simulink model "Speedmeter_harness"  (R2019b)
settings: Solver=FixedStepDiscrete  StartTime=0  StopTime=0.58999999999999997  FixedStep=0.01  RelTol=1e-3
undefined symbols (not defined in the file): Const16_0, Const16_2, Const16_210, Const16_340, Const16_350, Const16_4, Const8_0, Const8_1, Const8_2, Const8_4, ConstFL_00879, ConstFL_01, ConstFL_03516, ConstFL_1_6093, sigbuilder_block, STEP_TIME
libraries: simulink x2
(part 1 of 2)
settings Model: DataTypeOverride=Single  SldvGeneratedHarnessModel=TestUnitModel=Speedmeter|  ModifiedByFormat=TATA ELXSI LTD  Creator=TATA ELXSI LTD  LastModifiedBy=TATA ELXSI LTD
settings ConfigSet: Description=Test1
settings DataIOCC: LimitDataPoints=on  SaveFormat=StructureWithTime  ReturnWorkspaceOutputs=off
settings OptimizationCC: BlockReduction=off  ExpressionFolding=off  LifeSpan=inf
settings DebuggingCC: UnderspecifiedInitializationDetection=Classic  MergeDetectMultiDrivingBlocksExec=none  SolverPrmCheckMsg=warning  InheritedTsInSrcMsg=none  ParameterPrecisionLossMsg=none  FcnCallInpInsideContextMsg=warning  StateNameClashWarn=warning  SFUnexpectedBacktrackingDiag=warning  SFNoUnconditionalDefaultTransitionDiag=warning  SFExecutionAtInitializationDiag=none
settings HardwareCC: ProdBitPerPointer=32  ProdBitPerSizeT=32  ProdBitPerPtrDiffT=32  ProdLargestAtomicFloat=None  ProdWordSize=32  ProdHWDeviceType=Generic->32-bit x86 compatible
settings ModelReferenceCC: PropagateSignalLabelsOutOfModel=off
settings RTWCC: Description=Generic Real-Time Target
settings CodeAppCC: StateflowObjectComments=on
settings GRTTargetCC: TargetLangStandard=C89/C90 (ANSI)  CombineOutputUpdateFcns=off  GRTInterface=on
settings ConfigComp: CovEnable=on  RecordCoverage=on  CovMetricSettings=dcmo  CovHTMLOptions=-aTS=1 -bRG=1 -bTC=0 -hTR=0 -nFC=0 -scm=1 -bcm=1  CovHtmlReporting=on  CovSaveCumulativeToWorkspaceVar=on  CovCumulativeReport=on  CovShowResultsExplorer=off  CovModelRefEnable=on  DVMaxTestCaseSteps=500  DVTestSuiteOptimization=CombinedObjectives (Nonlinear Extended)  DVDetectDeadLogic=on  DVDetectActiveLogic=on  DVDetectOutOfBounds=on

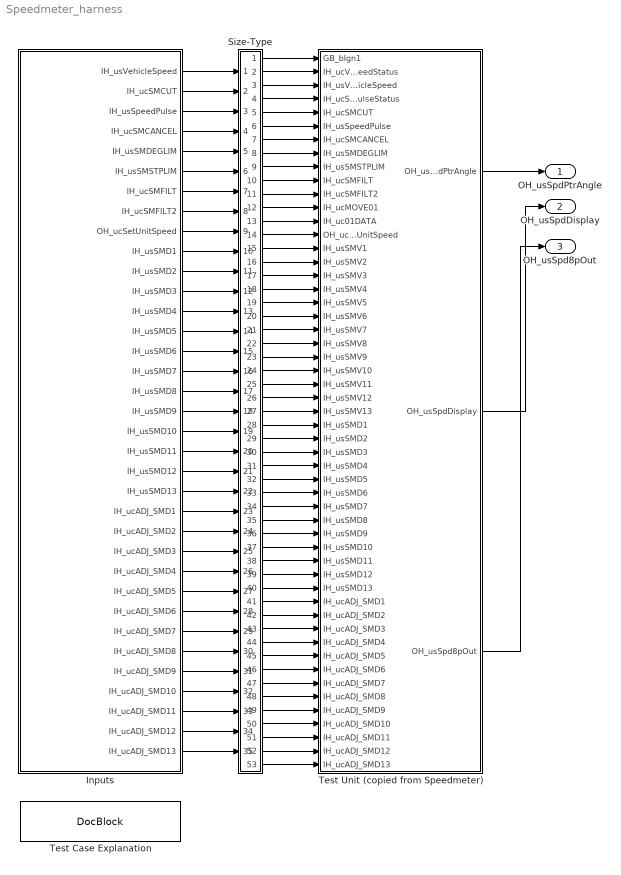
== system Speedmeter_harness ==
  Inputs : Subsystem  Tag=STV Subsys  LoadFcn=sigbuilder_block('load',[50 50 520 400 ]);  StartFcn=sigbuilder_block('start');  StopFcn=sigbuilder_block('stop');  ClipboardFcn=sigbuilder_block('clipboard');  mask(Sigbuilder block){tuvar=[0:10]}
      mask init:
      | if ~strcmp(get_param(bdroot(gcb),'SimulationStatus'),'stopped'),tuvar = sigbuilder_block('maskInit'); end
      settings: CopyFcn=sigbuilder_block('copy');  DeleteFcn=sigbuilder_block('delete');  ModelCloseFcn=sigbuilder_block('modelClose');  PreSaveFcn=sigbuilder_block('preSave');  PauseFcn=sigbuilder_block('pause');  ContinueFcn=sigbuilder_block('continue');  NameChangeFcn=sigbuilder_block('namechange');  OpenFcn=sigbuilder_block('open');  CloseFcn=sigbuilder_block('close');
      mask Display: plot(0, 0, 100, 100,[2, 2, 32, 32, 2], [68, 8, 8, 68, 68],[32, 2], [38, 38], [32, 19, 2],[53, 60, 44], [32, 17, 17, 2],[16, 16, 31, 31]);txt = getActiveGroup(gcbh);text(2, 100, txt,'verticalAlignment', 'top');
  Size-Type : Subsystem
  Test Case Explanation : simulink/Model-Wide Utilities/DocBlock  DocumentType=Text
  Test Unit (copied from Speedmeter) : Subsystem
  OH_usSpdPtrAngle : Outport  OutMin=0  OutMax=4095  OutDataTypeStr=fixdt(0,16,0.0879,0)  SampleTime=STEP_TIME  VectorParamsAs1DForOutWhenUnconnected=off
  OH_usSpdDisplay : Outport  Port=2  OutDataTypeStr=fixdt(0,16,1,0)  SampleTime=STEP_TIME  VectorParamsAs1DForOutWhenUnconnected=off
  OH_usSpd8pOut : Outport  Port=3  OutMin=0  OutMax=655.34  OutDataTypeStr=fixdt(0,16,0.01,0)  SampleTime=STEP_TIME  VectorParamsAs1DForOutWhenUnconnected=off
  wires:
  Size-Type/1(Out1) -> Test Unit (copied from Speedmeter)/1(GB_bIgn1)
  Size-Type/2(Out2) -> Test Unit (copied from Speedmeter)/2(IH_ucVehicleSpeedStatus)
  Inputs/1(IH_usVehicleSpeed) -> Size-Type/1(In3)
  Size-Type/3(Out3) -> Test Unit (copied from Speedmeter)/3(IH_usVehicleSpeed)
  Size-Type/4(Out4) -> Test Unit (copied from Speedmeter)/4(IH_ucSpeedPulseStatus)
  Inputs/2(IH_ucSMCUT) -> Size-Type/2(In5)
  Size-Type/5(Out5) -> Test Unit (copied from Speedmeter)/5(IH_ucSMCUT)
  Inputs/3(IH_usSpeedPulse) -> Size-Type/3(In6)
  Size-Type/6(Out6) -> Test Unit (copied from Speedmeter)/6(IH_usSpeedPulse)
  Inputs/4(IH_ucSMCANCEL) -> Size-Type/4(In7)
  Size-Type/7(Out7) -> Test Unit (copied from Speedmeter)/7(IH_ucSMCANCEL)
  Inputs/5(IH_usSMDEGLIM) -> Size-Type/5(In8)
  Size-Type/8(Out8) -> Test Unit (copied from Speedmeter)/8(IH_usSMDEGLIM)
  Inputs/6(IH_usSMSTPLIM) -> Size-Type/6(In9)
  Size-Type/9(Out9) -> Test Unit (copied from Speedmeter)/9(IH_usSMSTPLIM)
  Inputs/7(IH_ucSMFILT) -> Size-Type/7(In10)
  Size-Type/10(Out10) -> Test Unit (copied from Speedmeter)/10(IH_ucSMFILT)
  Inputs/8(IH_ucSMFILT2) -> Size-Type/8(In11)
  Size-Type/11(Out11) -> Test Unit (copied from Speedmeter)/11(IH_ucSMFILT2)
  Size-Type/12(Out12) -> Test Unit (copied from Speedmeter)/12(IH_ucMOVE01)
  Size-Type/13(Out13) -> Test Unit (copied from Speedmeter)/13(IH_uc01DATA)
  Inputs/9(OH_ucSetUnitSpeed) -> Size-Type/9(In14)
  Size-Type/14(Out14) -> Test Unit (copied from Speedmeter)/14(OH_ucSetUnitSpeed)
  Size-Type/15(Out15) -> Test Unit (copied from Speedmeter)/15(IH_usSMV1)
  Size-Type/16(Out16) -> Test Unit (copied from Speedmeter)/16(IH_usSMV2)
  Size-Type/17(Out17) -> Test Unit (copied from Speedmeter)/17(IH_usSMV3)
  Size-Type/18(Out18) -> Test Unit (copied from Speedmeter)/18(IH_usSMV4)
  Size-Type/19(Out19) -> Test Unit (copied from Speedmeter)/19(IH_usSMV5)
  Size-Type/20(Out20) -> Test Unit (copied from Speedmeter)/20(IH_usSMV6)
  Size-Type/21(Out21) -> Test Unit (copied from Speedmeter)/21(IH_usSMV7)
  Size-Type/22(Out22) -> Test Unit (copied from Speedmeter)/22(IH_usSMV8)
  Size-Type/23(Out23) -> Test Unit (copied from Speedmeter)/23(IH_usSMV9)
  Size-Type/24(Out24) -> Test Unit (copied from Speedmeter)/24(IH_usSMV10)
  Size-Type/25(Out25) -> Test Unit (copied from Speedmeter)/25(IH_usSMV11)
  Size-Type/26(Out26) -> Test Unit (copied from Speedmeter)/26(IH_usSMV12)
  Size-Type/27(Out27) -> Test Unit (copied from Speedmeter)/27(IH_usSMV13)
  Inputs/10(IH_usSMD1) -> Size-Type/10(In28)
  Size-Type/28(Out28) -> Test Unit (copied from Speedmeter)/28(IH_usSMD1)
  Inputs/11(IH_usSMD2) -> Size-Type/11(In29)
  Size-Type/29(Out29) -> Test Unit (copied from Speedmeter)/29(IH_usSMD2)
  Inputs/12(IH_usSMD3) -> Size-Type/12(In30)
  Size-Type/30(Out30) -> Test Unit (copied from Speedmeter)/30(IH_usSMD3)
  Inputs/13(IH_usSMD4) -> Size-Type/13(In31)
  Size-Type/31(Out31) -> Test Unit (copied from Speedmeter)/31(IH_usSMD4)
  Inputs/14(IH_usSMD5) -> Size-Type/14(In32)
  Size-Type/32(Out32) -> Test Unit (copied from Speedmeter)/32(IH_usSMD5)
  Inputs/15(IH_usSMD6) -> Size-Type/15(In33)
  Size-Type/33(Out33) -> Test Unit (copied from Speedmeter)/33(IH_usSMD6)
  Inputs/16(IH_usSMD7) -> Size-Type/16(In34)
  Size-Type/34(Out34) -> Test Unit (copied from Speedmeter)/34(IH_usSMD7)
  Inputs/17(IH_usSMD8) -> Size-Type/17(In35)
  Size-Type/35(Out35) -> Test Unit (copied from Speedmeter)/35(IH_usSMD8)
  Inputs/18(IH_usSMD9) -> Size-Type/18(In36)
  Size-Type/36(Out36) -> Test Unit (copied from Speedmeter)/36(IH_usSMD9)
  Inputs/19(IH_usSMD10) -> Size-Type/19(In37)
  Size-Type/37(Out37) -> Test Unit (copied from Speedmeter)/37(IH_usSMD10)
  Inputs/20(IH_usSMD11) -> Size-Type/20(In38)
  Size-Type/38(Out38) -> Test Unit (copied from Speedmeter)/38(IH_usSMD11)
  Inputs/21(IH_usSMD12) -> Size-Type/21(In39)
  Size-Type/39(Out39) -> Test Unit (copied from Speedmeter)/39(IH_usSMD12)
  Inputs/22(IH_usSMD13) -> Size-Type/22(In40)
  Size-Type/40(Out40) -> Test Unit (copied from Speedmeter)/40(IH_usSMD13)
  Inputs/23(IH_ucADJ_SMD1) -> Size-Type/23(In41)
  Size-Type/41(Out41) -> Test Unit (copied from Speedmeter)/41(IH_ucADJ_SMD1)
  Inputs/24(IH_ucADJ_SMD2) -> Size-Type/24(In42)
  Size-Type/42(Out42) -> Test Unit (copied from Speedmeter)/42(IH_ucADJ_SMD2)
  Inputs/25(IH_ucADJ_SMD3) -> Size-Type/25(In43)
  Size-Type/43(Out43) -> Test Unit (copied from Speedmeter)/43(IH_ucADJ_SMD3)
  Inputs/26(IH_ucADJ_SMD4) -> Size-Type/26(In44)
  Size-Type/44(Out44) -> Test Unit (copied from Speedmeter)/44(IH_ucADJ_SMD4)
  Inputs/27(IH_ucADJ_SMD5) -> Size-Type/27(In45)
  Size-Type/45(Out45) -> Test Unit (copied from Speedmeter)/45(IH_ucADJ_SMD5)
  Inputs/28(IH_ucADJ_SMD6) -> Size-Type/28(In46)
  Size-Type/46(Out46) -> Test Unit (copied from Speedmeter)/46(IH_ucADJ_SMD6)
  Inputs/29(IH_ucADJ_SMD7) -> Size-Type/29(In47)
  Size-Type/47(Out47) -> Test Unit (copied from Speedmeter)/47(IH_ucADJ_SMD7)
  Inputs/30(IH_ucADJ_SMD8) -> Size-Type/30(In48)
  Size-Type/48(Out48) -> Test Unit (copied from Speedmeter)/48(IH_ucADJ_SMD8)
  Inputs/31(IH_ucADJ_SMD9) -> Size-Type/31(In49)
  Size-Type/49(Out49) -> Test Unit (copied from Speedmeter)/49(IH_ucADJ_SMD9)
  Inputs/32(IH_ucADJ_SMD10) -> Size-Type/32(In50)
  Size-Type/50(Out50) -> Test Unit (copied from Speedmeter)/50(IH_ucADJ_SMD10)
  Inputs/33(IH_ucADJ_SMD11) -> Size-Type/33(In51)
  Size-Type/51(Out51) -> Test Unit (copied from Speedmeter)/51(IH_ucADJ_SMD11)
  Inputs/34(IH_ucADJ_SMD12) -> Size-Type/34(In52)
  Size-Type/52(Out52) -> Test Unit (copied from Speedmeter)/52(IH_ucADJ_SMD12)
  Inputs/35(IH_ucADJ_SMD13) -> Size-Type/35(In53)
  Size-Type/53(Out53) -> Test Unit (copied from Speedmeter)/53(IH_ucADJ_SMD13)
  Test Unit (copied from Speedmeter)/1(OH_usSpdPtrAngle) -> OH_usSpdPtrAngle/1
  Test Unit (copied from Speedmeter)/2(OH_usSpdDisplay) -> OH_usSpdDisplay/1
  Test Unit (copied from Speedmeter)/3(OH_usSpd8pOut) -> OH_usSpd8pOut/1

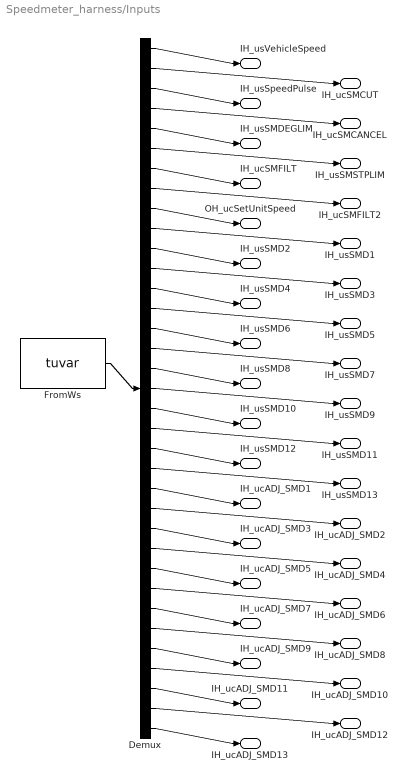
== system Speedmeter_harness/Inputs ==
  Demux : Demux  Tag=STV Demux  Outputs=35
  FromWs : FromWorkspace  Tag=STV FromWs  VariableName=tuvar  SampleTime=0
      SigBuilderData=|
      | dataSet.timeRange = [0 2.38]
      | dataSet.name = 'Test Case 1'
      | sbobj.Name = 'Signal Builder'
      | sbobj.Groups.Name = 'Test Case 1'
      | sbobj.Groups.Signals(1).Name = 'IH_usVehicleSpeed'
      | sbobj.Groups.Signals(1).XData = [0 2.18 2.18 2.21 2.23 2.35 2.36 2.37 2.38]
      | sbobj.Groups.Signals(1).YData = [404.191131592 404.191131592 0 0 0 0 0 0 0]
      | sbobj.Groups.Signals(2).Name = 'IH_ucSMCUT'
      | sbobj.Groups.Signals(2).XData = [0 2.18 2.18 2.21 2.23 2.35 2.36 2.37 2.38]
      | sbobj.Groups.Signals(2).YData = [1.79223001003 1.79223001003 0 0 0 0 0 0 0]
      | sbobj.Groups.Signals(3).Name = 'IH_usSpeedPulse'
      | sbobj.Groups.Signals(3).XData = [0 2.18 2.18 2.21 2.21 2.23 2.23 2.35 2.35 2.36 2.36 2.37 2.38]
      | sbobj.Groups.Signals(3).YData = [320.146972656 320.146972656 0 0 655.349975586 655.349975586 0 0 655.349975586 655.349975586 0 0 0]
      | sbobj.Groups.Signals(4).Name = 'IH_ucSMCANCEL'
      | sbobj.Groups.Signals(4).XData = [0 2.18 2.18 2.21 2.23 2.35 2.36 2.37 2.37 2.38]
      | sbobj.Groups.Signals(4).YData = [1.19769001007 1.19769001007 0 0 0 0 0 0 10.899600029 10.899600029]
      | sbobj.Groups.Signals(5).Name = 'IH_usSMDEGLIM'
      | sbobj.Groups.Signals(5).XData = [0 2.18 2.21 2.23 2.35 2.35 2.36 2.36 2.37 2.38]
      | sbobj.Groups.Signals(5).YData = [140.597106934 140.597106934 140.597106934 140.597106934 140.597106934 82.1601867676 82.1601867676 0 0 0]
      | sbobj.Groups.Signals(6).Name = 'IH_usSMSTPLIM'
      | sbobj.Groups.Signals(6).XData = [0 2.18 2.18 2.21 2.23 2.35 2.35 2.36 2.37 2.38]
      | sbobj.Groups.Signals(6).YData = [0.951390028 0.951390028 5.53770017624 5.53770017624 5.53770017624 5.53770017624 0 0 0 0]
      | sbobj.Groups.Signals(7).Name = 'IH_ucSMFILT'
      | sbobj.Groups.Signals(7).XData = [0 2.18 2.21 2.23 2.35 2.36 2.37 2.37 2.38]
      | sbobj.Groups.Signals(7).YData = [4.00516986847 4.00516986847 4.00516986847 4.00516986847 4.00516986847 4.00516986847 4.00516986847 0 0]
      | sbobj.Groups.Signals(8).Name = 'IH_ucSMFILT2'
      | sbobj.Groups.Signals(8).XData = [0 2.18 2.21 2.23 2.35 2.36 2.37 2.37 2.38]
      | sbobj.Groups.Signals(8).YData = [1.31280994415 1.31280994415 1.31280994415 1.31280994415 1.31280994415 1.31280994415 1.31280994415 0 0]
      | sbobj.Groups.Signals(9).Name = 'OH_ucSetUnitSpeed'
      | sbobj.Groups.Signals(9).XData = [0 2.18 2.18 2.21 2.23 2.23 2.35 2.36 2.36 2.37 2.38]
      | sbobj.Groups.Signals(9).YData = [0.490040004253 0.490040004253 0 0 0 1 1 1 0 0 0]
      | sbobj.Groups.Signals(10).Name = 'IH_usSMD1'
      | sbobj.Groups.Signals(10).XData = [0 2.18 2.18 2.21 2.23 2.35 2.36 2.37 2.38]
      | sbobj.Groups.Signals(10).YData = [192.551025391 192.551025391 0 0 0 0 0 0 0]
      | sbobj.Groups.Signals(11).Name = 'IH_usSMD2'
      | sbobj.Groups.Signals(11).XData = [0 2.18 2.18 2.21 2.23 2.35 2.35 2.36 2.36 2.37 2.38]
      | sbobj.Groups.Signals(11).YData = [115.773422241 115.773422241 0 0 0 0 359.950500488 359.950500488 0 0 0]
      | sbobj.Groups.Signals(12).Name = 'IH_usSMD3'
      | sbobj.Groups.Signals(12).XData = [0 2.18 2.18 2.21 2.23 2.35 2.35 2.36 2.36 2.37 2.38]
      | sbobj.Groups.Signals(12).YData = [191.705841064 191.705841064 0 0 0 0 359.950500488 359.950500488 0 0 0]
      | sbobj.Groups.Signals(13).Name = 'IH_usSMD4'
      | sbobj.Groups.Signals(13).XData = [0 2.18 2.18 2.21 2.23 2.35 2.35 2.36 2.36 2.37 2.38]
      | sbobj.Groups.Signals(13).YData = [73.4985580444 73.4985580444 0 0 0 0 359.950500488 359.950500488 0 0 0]
      | sbobj.Groups.Signals(14).Name = 'IH_usSMD5'
      | sbobj.Groups.Signals(14).XData = [0 2.18 2.18 2.21 2.23 2.35 2.35 2.36 2.36 2.37 2.38]
      | sbobj.Groups.Signals(14).YData = [124.571632385 124.571632385 0 0 0 0 359.950500488 359.950500488 0 0 0]
      | sbobj.Groups.Signals(15).Name = 'IH_usSMD6'
      | sbobj.Groups.Signals(15).XData = [0 2.18 2.18 2.21 2.23 2.35 2.35 2.36 2.36 2.37 2.38]
      | sbobj.Groups.Signals(15).YData = [180.208282471 180.208282471 0 0 0 0 359.950500488 359.950500488 0 0 0]
      | sbobj.Groups.Signals(16).Name = 'IH_usSMD7'
      | sbobj.Groups.Signals(16).XData = [0 2.18 2.18 2.21 2.23 2.35 2.35 2.36 2.36 2.37 2.38]
      | sbobj.Groups.Signals(16).YData = [189.461975098 189.461975098 0 0 0 0 359.950500488 359.950500488 0 0 0]
      | sbobj.Groups.Signals(17).Name = 'IH_usSMD8'
      | sbobj.Groups.Signals(17).XData = [0 2.18 2.18 2.21 2.23 2.35 2.35 2.36 2.36 2.37 2.38]
      | sbobj.Groups.Signals(17).YData = [84.5667572021 84.5667572021 0 0 0 0 359.950500488 359.950500488 0 0 0]
      | sbobj.Groups.Signals(18).Name = 'IH_usSMD9'
      | sbobj.Groups.Signals(18).XData = [0 2.18 2.18 2.21 2.23 2.35 2.35 2.36 2.36 2.37 2.38]
      | sbobj.Groups.Signals(18).YData = [196.988327026 196.988327026 0 0 0 0 359.950500488 359.950500488 0 0 0]
      | sbobj.Groups.Signals(19).Name = 'IH_usSMD10'
      | sbobj.Groups.Signals(19).XData = [0 2.18 2.18 2.21 2.23 2.35 2.35 2.36 2.36 2.37 2.38]
      | sbobj.Groups.Signals(19).YData = [206.035125732 206.035125732 0 0 0 0 359.950500488 359.950500488 0 0 0]
      | sbobj.Groups.Signals(20).Name = 'IH_usSMD11'
      | sbobj.Groups.Signals(20).XData = [0 2.18 2.18 2.21 2.23 2.35 2.35 2.36 2.36 2.37 2.38]
      | sbobj.Groups.Signals(20).YData = [305.747680664 305.747680664 0 0 0 0 359.950500488 359.950500488 0 0 0]
      | sbobj.Groups.Signals(21).Name = 'IH_usSMD12'
      | sbobj.Groups.Signals(21).XData = [0 2.18 2.18 2.21 2.23 2.35 2.35 2.36 2.36 2.37 2.38]
      | sbobj.Groups.Signals(21).YData = [10.1902399063 10.1902399063 0 0 0 0 359.950500488 359.950500488 0 0 0]
      | sbobj.Groups.Signals(22).Name = 'IH_usSMD13'
      | sbobj.Groups.Signals(22).XData = [0 2.18 2.18 2.21 2.23 2.35 2.35 2.36 2.36 2.37 2.38]
      | sbobj.Groups.Signals(22).YData = [147.716644287 147.716644287 0.140892744064 0.140892744064 0.140892744064 0.140892744064 359.950500488 359.950500488 0 0 0]
      | sbobj.Groups.Signals(23).Name = 'IH_ucADJ_SMD1'
      | sbobj.Groups.Signals(23).XData = [0 2.18 2.18 2.21 2.23 2.35 2.36 2.37 2.38]
      | sbobj.Groups.Signals(23).YData = [7.73224020004 7.73224020004 0 0 0 0 0 0 0]
      | sbobj.Groups.Signals(24).Name = 'IH_ucADJ_SMD2'
      | sbobj.Groups.Signals(24).XData = [0 2.18 2.18 2.21 2.23 2.35 2.35 2.36 2.36 2.37 2.38]
      | sbobj.Groups.Signals(24).YData = [16.1306705475 16.1306705475 0 0 0 0 22.4144992828 22.4144992828 0 0 0]
      | sbobj.Groups.Signals(25).Name = 'IH_ucADJ_SMD3'
      | sbobj.Groups.Signals(25).XData = [0 2.18 2.18 2.21 2.23 2.35 2.35 2.36 2.36 2.37 2.38]
      | sbobj.Groups.Signals(25).YData = [9.09510993958 9.09510993958 0 0 0 0 22.4144992828 22.4144992828 0 0 0]
      | sbobj.Groups.Signals(26).Name = 'IH_ucADJ_SMD4'
      | sbobj.Groups.Signals(26).XData = [0 2.18 2.18 2.21 2.23 2.35 2.35 2.36 2.36 2.37 2.38]
      | sbobj.Groups.Signals(26).YData = [18.9658699036 18.9658699036 0 0 0 0 22.4144992828 22.4144992828 0 0 0]
      | sbobj.Groups.Signals(27).Name = 'IH_ucADJ_SMD5'
      | sbobj.Groups.Signals(27).XData = [0 2.18 2.18 2.21 2.23 2.35 2.35 2.36 2.36 2.37 2.38]
      | sbobj.Groups.Signals(27).YData = [19.2279605865 19.2279605865 0 0 0 0 22.4144992828 22.4144992828 0 0 0]
      | sbobj.Groups.Signals(28).Name = 'IH_ucADJ_SMD6'
      | sbobj.Groups.Signals(28).XData = [0 2.18 2.18 2.21 2.23 2.35 2.35 2.36 2.36 2.37 2.38]
      | sbobj.Groups.Signals(28).YData = [0.32798999548 0.32798999548 0 0 0 0 22.4144992828 22.4144992828 0 0 0]
      | sbobj.Groups.Signals(29).Name = 'IH_ucADJ_SMD7'
      | sbobj.Groups.Signals(29).XData = [0 2.18 2.18 2.21 2.23 2.35 2.35 2.36 2.36 2.37 2.38]
      | sbobj.Groups.Signals(29).YData = [0.398829996586 0.398829996586 0 0 0 0 22.4144992828 22.4144992828 0 0 0]
      | sbobj.Groups.Signals(30).Name = 'IH_ucADJ_SMD8'
      | sbobj.Groups.Signals(30).XData = [0 2.18 2.18 2.21 2.23 2.35 2.35 2.36 2.36 2.37 2.38]
      | sbobj.Groups.Signals(30).YData = [19.1637992859 19.1637992859 0 0 0 0 22.4144992828 22.4144992828 0 0 0]
      | sbobj.Groups.Signals(31).Name = 'IH_ucADJ_SMD9'
      | sbobj.Groups.Signals(31).XData = [0 2.18 2.18 2.21 2.23 2.35 2.35 2.36 2.36 2.37 2.38]
      | sbobj.Groups.Signals(31).YData = [2.60408997536 2.60408997536 0 0 0 0 22.4144992828 22.4144992828 0 0 0]
      | sbobj.Groups.Signals(32).Name = 'IH_ucADJ_SMD10'
      | sbobj.Groups.Signals(32).XData = [0 2.18 2.18 2.21 2.23 2.35 2.35 2.36 2.36 2.37 2.38]
      | sbobj.Groups.Signals(32).YData = [12.0242204666 12.0242204666 0 0 0 0 22.4144992828 22.4144992828 0 0 0]
      | sbobj.Groups.Signals(33).Name = 'IH_ucADJ_SMD11'
      | sbobj.Groups.Signals(33).XData = [0 2.18 2.18 2.21 2.23 2.35 2.35 2.36 2.36 2.37 2.38]
      | sbobj.Groups.Signals(33).YData = [5.76280021667 5.76280021667 0 0 0 0 22.4144992828 22.4144992828 0 0 0]
      | sbobj.Groups.Signals(34).Name = 'IH_ucADJ_SMD12'
      | sbobj.Groups.Signals(34).XData = [0 2.18 2.18 2.21 2.23 2.35 2.35 2.36 2.36 2.37 2.38]
      | sbobj.Groups.Signals(34).YData = [18.479839325 18.479839325 0 0 0 0 22.4144992828 22.4144992828 0 0 0]
      | sbobj.Groups.Signals(35).Name = 'IH_ucADJ_SMD13'
      | sbobj.Groups.Signals(35).XData = [0 2.18 2.18 2.21 2.23 2.35 2.35 2.36 2.36 2.37 2.38]
      | sbobj.Groups.Signals(35).YData = [8.36791038513 8.36791038513 0 0 0 0 22.4144992828 22.4144992828 0 0 0]
      | sbobj.Groups.TimeRange = [0 2.38]
  IH_usVehicleSpeed : Outport  Tag=STV Outport
  IH_ucSMCUT : Outport  Tag=STV Outport  Port=2
  IH_usSpeedPulse : Outport  Tag=STV Outport  Port=3
  IH_ucSMCANCEL : Outport  Tag=STV Outport  Port=4
  IH_usSMDEGLIM : Outport  Tag=STV Outport  Port=5
  IH_usSMSTPLIM : Outport  Tag=STV Outport  Port=6
  IH_ucSMFILT : Outport  Tag=STV Outport  Port=7
  IH_ucSMFILT2 : Outport  Tag=STV Outport  Port=8
  OH_ucSetUnitSpeed : Outport  Tag=STV Outport  Port=9
  IH_usSMD1 : Outport  Tag=STV Outport  Port=10
  IH_usSMD2 : Outport  Tag=STV Outport  Port=11
  IH_usSMD3 : Outport  Tag=STV Outport  Port=12
  IH_usSMD4 : Outport  Tag=STV Outport  Port=13
  IH_usSMD5 : Outport  Tag=STV Outport  Port=14
  IH_usSMD6 : Outport  Tag=STV Outport  Port=15
  IH_usSMD7 : Outport  Tag=STV Outport  Port=16
  IH_usSMD8 : Outport  Tag=STV Outport  Port=17
  IH_usSMD9 : Outport  Tag=STV Outport  Port=18
  IH_usSMD10 : Outport  Tag=STV Outport  Port=19
  IH_usSMD11 : Outport  Tag=STV Outport  Port=20
  IH_usSMD12 : Outport  Tag=STV Outport  Port=21
  IH_usSMD13 : Outport  Tag=STV Outport  Port=22
  IH_ucADJ_SMD1 : Outport  Tag=STV Outport  Port=23
  IH_ucADJ_SMD2 : Outport  Tag=STV Outport  Port=24
  IH_ucADJ_SMD3 : Outport  Tag=STV Outport  Port=25
  IH_ucADJ_SMD4 : Outport  Tag=STV Outport  Port=26
  IH_ucADJ_SMD5 : Outport  Tag=STV Outport  Port=27
  IH_ucADJ_SMD6 : Outport  Tag=STV Outport  Port=28
  IH_ucADJ_SMD7 : Outport  Tag=STV Outport  Port=29
  IH_ucADJ_SMD8 : Outport  Tag=STV Outport  Port=30
  IH_ucADJ_SMD9 : Outport  Tag=STV Outport  Port=31
  IH_ucADJ_SMD10 : Outport  Tag=STV Outport  Port=32
  IH_ucADJ_SMD11 : Outport  Tag=STV Outport  Port=33
  IH_ucADJ_SMD12 : Outport  Tag=STV Outport  Port=34
  IH_ucADJ_SMD13 : Outport  Tag=STV Outport  Port=35
  wires:
  FromWs/1 -> Demux/1
  Demux/1 -> IH_usVehicleSpeed/1
  Demux/2 -> IH_ucSMCUT/1
  Demux/3 -> IH_usSpeedPulse/1
  Demux/4 -> IH_ucSMCANCEL/1
  Demux/5 -> IH_usSMDEGLIM/1
  Demux/6 -> IH_usSMSTPLIM/1
  Demux/7 -> IH_ucSMFILT/1
  Demux/8 -> IH_ucSMFILT2/1
  Demux/9 -> OH_ucSetUnitSpeed/1
  Demux/10 -> IH_usSMD1/1
  Demux/11 -> IH_usSMD2/1
  Demux/12 -> IH_usSMD3/1
  Demux/13 -> IH_usSMD4/1
  Demux/14 -> IH_usSMD5/1
  Demux/15 -> IH_usSMD6/1
  Demux/16 -> IH_usSMD7/1
  Demux/17 -> IH_usSMD8/1
  Demux/18 -> IH_usSMD9/1
  Demux/19 -> IH_usSMD10/1
  Demux/20 -> IH_usSMD11/1
  Demux/21 -> IH_usSMD12/1
  Demux/22 -> IH_usSMD13/1
  Demux/23 -> IH_ucADJ_SMD1/1
  Demux/24 -> IH_ucADJ_SMD2/1
  Demux/25 -> IH_ucADJ_SMD3/1
  Demux/26 -> IH_ucADJ_SMD4/1
  Demux/27 -> IH_ucADJ_SMD5/1
  Demux/28 -> IH_ucADJ_SMD6/1
  Demux/29 -> IH_ucADJ_SMD7/1
  Demux/30 -> IH_ucADJ_SMD8/1
  Demux/31 -> IH_ucADJ_SMD9/1
  Demux/32 -> IH_ucADJ_SMD10/1
  Demux/33 -> IH_ucADJ_SMD11/1
  Demux/34 -> IH_ucADJ_SMD12/1
  Demux/35 -> IH_ucADJ_SMD13/1

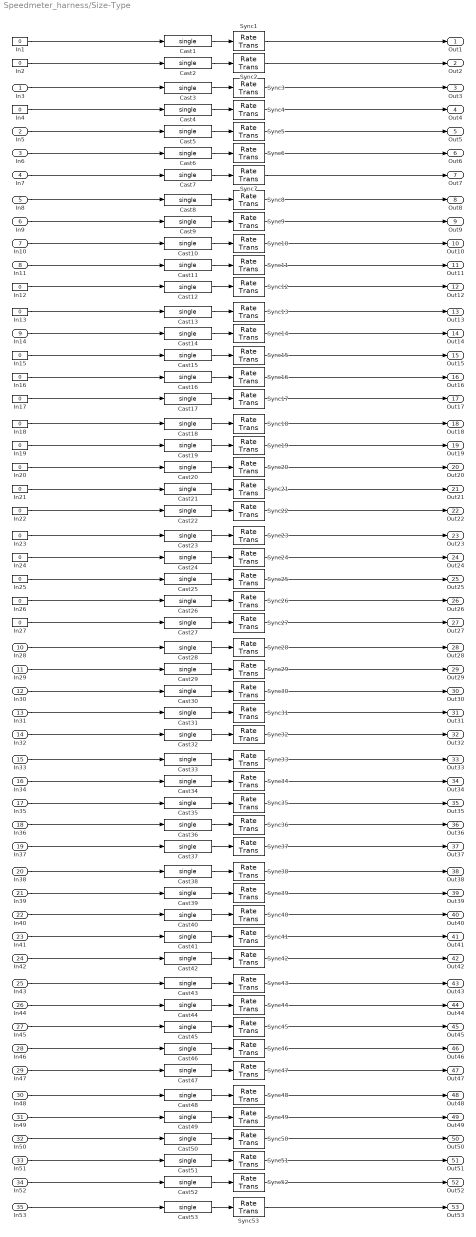
== system Speedmeter_harness/Size-Type ==
  In3 : Inport
  In5 : Inport  Port=2
  In6 : Inport  Port=3
  In7 : Inport  Port=4
  In8 : Inport  Port=5
  In9 : Inport  Port=6
  In10 : Inport  Port=7
  In11 : Inport  Port=8
  In14 : Inport  Port=9
  In28 : Inport  Port=10
  In29 : Inport  Port=11
  In30 : Inport  Port=12
  In31 : Inport  Port=13
  In32 : Inport  Port=14
  In33 : Inport  Port=15
  In34 : Inport  Port=16
  In35 : Inport  Port=17
  In36 : Inport  Port=18
  In37 : Inport  Port=19
  In38 : Inport  Port=20
  In39 : Inport  Port=21
  In40 : Inport  Port=22
  In41 : Inport  Port=23
  In42 : Inport  Port=24
  In43 : Inport  Port=25
  In44 : Inport  Port=26
  In45 : Inport  Port=27
  In46 : Inport  Port=28
  In47 : Inport  Port=29
  In48 : Inport  Port=30
  In49 : Inport  Port=31
  In50 : Inport  Port=32
  In51 : Inport  Port=33
  In52 : Inport  Port=34
  In53 : Inport  Port=35
  Cast{1..53} (53 alike) : DataTypeConversion  OutDataTypeStr=single  RndMeth=Nearest  SaturateOnIntegerOverflow=on
  In{1..2,4,12..13,15..27} (18 alike) : Constant  Value=0  OutDataTypeStr=double
  Sync{1..53} (53 alike) : RateTransition  OutPortSampleTime=[0.01,0]
  Out1 : Outport
  Out2 : Outport  Port=2
  Out3 : Outport  Port=3
  Out4 : Outport  Port=4
  Out5 : Outport  Port=5
  Out6 : Outport  Port=6
  Out7 : Outport  Port=7
  Out8 : Outport  Port=8
  Out9 : Outport  Port=9
  Out10 : Outport  Port=10
  Out11 : Outport  Port=11
  Out12 : Outport  Port=12
  Out13 : Outport  Port=13
  Out14 : Outport  Port=14
  Out15 : Outport  Port=15
  Out16 : Outport  Port=16
  Out17 : Outport  Port=17
  Out18 : Outport  Port=18
  Out19 : Outport  Port=19
  Out20 : Outport  Port=20
  Out21 : Outport  Port=21
  Out22 : Outport  Port=22
  Out23 : Outport  Port=23
  Out24 : Outport  Port=24
  Out25 : Outport  Port=25
  Out26 : Outport  Port=26
  Out27 : Outport  Port=27
  Out28 : Outport  Port=28
  Out29 : Outport  Port=29
  Out30 : Outport  Port=30
  Out31 : Outport  Port=31
  Out32 : Outport  Port=32
  Out33 : Outport  Port=33
  Out34 : Outport  Port=34
  Out35 : Outport  Port=35
  Out36 : Outport  Port=36
  Out37 : Outport  Port=37
  Out38 : Outport  Port=38
  Out39 : Outport  Port=39
  Out40 : Outport  Port=40
  Out41 : Outport  Port=41
  Out42 : Outport  Port=42
  Out43 : Outport  Port=43
  Out44 : Outport  Port=44
  Out45 : Outport  Port=45
  Out46 : Outport  Port=46
  Out47 : Outport  Port=47
  Out48 : Outport  Port=48
  Out49 : Outport  Port=49
  Out50 : Outport  Port=50
  Out51 : Outport  Port=51
  Out52 : Outport  Port=52
  Out53 : Outport  Port=53
  wires:
  In1/1 -> Cast1/1
  Cast1/1 -> Sync1/1
  Sync1/1 -> Out1/1
  In2/1 -> Cast2/1
  Cast2/1 -> Sync2/1
  Sync2/1 -> Out2/1
  In3/1 -> Cast3/1
  Cast3/1 -> Sync3/1
  Sync3/1 -> Out3/1
  In4/1 -> Cast4/1
  Cast4/1 -> Sync4/1
  Sync4/1 -> Out4/1
  In5/1 -> Cast5/1
  Cast5/1 -> Sync5/1
  Sync5/1 -> Out5/1
  In6/1 -> Cast6/1
  Cast6/1 -> Sync6/1
  Sync6/1 -> Out6/1
  In7/1 -> Cast7/1
  Cast7/1 -> Sync7/1
  Sync7/1 -> Out7/1
  In8/1 -> Cast8/1
  Cast8/1 -> Sync8/1
  Sync8/1 -> Out8/1
  In9/1 -> Cast9/1
  Cast9/1 -> Sync9/1
  Sync9/1 -> Out9/1
  In10/1 -> Cast10/1
  Cast10/1 -> Sync10/1
  Sync10/1 -> Out10/1
  In11/1 -> Cast11/1
  Cast11/1 -> Sync11/1
  Sync11/1 -> Out11/1
  In12/1 -> Cast12/1
  Cast12/1 -> Sync12/1
  Sync12/1 -> Out12/1
  In13/1 -> Cast13/1
  Cast13/1 -> Sync13/1
  Sync13/1 -> Out13/1
  In14/1 -> Cast14/1
  Cast14/1 -> Sync14/1
  Sync14/1 -> Out14/1
  In15/1 -> Cast15/1
  Cast15/1 -> Sync15/1
  Sync15/1 -> Out15/1
  In16/1 -> Cast16/1
  Cast16/1 -> Sync16/1
  Sync16/1 -> Out16/1
  In17/1 -> Cast17/1
  Cast17/1 -> Sync17/1
  Sync17/1 -> Out17/1
  In18/1 -> Cast18/1
  Cast18/1 -> Sync18/1
  Sync18/1 -> Out18/1
  In19/1 -> Cast19/1
  Cast19/1 -> Sync19/1
  Sync19/1 -> Out19/1
  In20/1 -> Cast20/1
  Cast20/1 -> Sync20/1
  Sync20/1 -> Out20/1
  In21/1 -> Cast21/1
  Cast21/1 -> Sync21/1
  Sync21/1 -> Out21/1
  In22/1 -> Cast22/1
  Cast22/1 -> Sync22/1
  Sync22/1 -> Out22/1
  In23/1 -> Cast23/1
  Cast23/1 -> Sync23/1
  Sync23/1 -> Out23/1
  In24/1 -> Cast24/1
  Cast24/1 -> Sync24/1
  Sync24/1 -> Out24/1
  In25/1 -> Cast25/1
  Cast25/1 -> Sync25/1
  Sync25/1 -> Out25/1
  In26/1 -> Cast26/1
  Cast26/1 -> Sync26/1
  Sync26/1 -> Out26/1
  In27/1 -> Cast27/1
  Cast27/1 -> Sync27/1
  Sync27/1 -> Out27/1
  In28/1 -> Cast28/1
  Cast28/1 -> Sync28/1
  Sync28/1 -> Out28/1
  In29/1 -> Cast29/1
  Cast29/1 -> Sync29/1
  Sync29/1 -> Out29/1
  In30/1 -> Cast30/1
  Cast30/1 -> Sync30/1
  Sync30/1 -> Out30/1
  In31/1 -> Cast31/1
  Cast31/1 -> Sync31/1
  Sync31/1 -> Out31/1
  In32/1 -> Cast32/1
  Cast32/1 -> Sync32/1
  Sync32/1 -> Out32/1
  In33/1 -> Cast33/1
  Cast33/1 -> Sync33/1
  Sync33/1 -> Out33/1
  In34/1 -> Cast34/1
  Cast34/1 -> Sync34/1
  Sync34/1 -> Out34/1
  In35/1 -> Cast35/1
  Cast35/1 -> Sync35/1
  Sync35/1 -> Out35/1
  In36/1 -> Cast36/1
  Cast36/1 -> Sync36/1
  Sync36/1 -> Out36/1
  In37/1 -> Cast37/1
  Cast37/1 -> Sync37/1
  Sync37/1 -> Out37/1
  In38/1 -> Cast38/1
  Cast38/1 -> Sync38/1
  Sync38/1 -> Out38/1
  In39/1 -> Cast39/1
  Cast39/1 -> Sync39/1
  Sync39/1 -> Out39/1
  In40/1 -> Cast40/1
  Cast40/1 -> Sync40/1
  Sync40/1 -> Out40/1
  In41/1 -> Cast41/1
  Cast41/1 -> Sync41/1
  Sync41/1 -> Out41/1
  In42/1 -> Cast42/1
  Cast42/1 -> Sync42/1
  Sync42/1 -> Out42/1
  In43/1 -> Cast43/1
  Cast43/1 -> Sync43/1
  Sync43/1 -> Out43/1
  In44/1 -> Cast44/1
  Cast44/1 -> Sync44/1
  Sync44/1 -> Out44/1
  In45/1 -> Cast45/1
  Cast45/1 -> Sync45/1
  Sync45/1 -> Out45/1
  In46/1 -> Cast46/1
  Cast46/1 -> Sync46/1
  Sync46/1 -> Out46/1
  In47/1 -> Cast47/1
  Cast47/1 -> Sync47/1
  Sync47/1 -> Out47/1
  In48/1 -> Cast48/1
  Cast48/1 -> Sync48/1
  Sync48/1 -> Out48/1
  In49/1 -> Cast49/1
  Cast49/1 -> Sync49/1
  Sync49/1 -> Out49/1
  In50/1 -> Cast50/1
  Cast50/1 -> Sync50/1
  Sync50/1 -> Out50/1
  In51/1 -> Cast51/1
  Cast51/1 -> Sync51/1
  Sync51/1 -> Out51/1
  In52/1 -> Cast52/1
  Cast52/1 -> Sync52/1
  Sync52/1 -> Out52/1
  In53/1 -> Cast53/1
  Cast53/1 -> Sync53/1
  Sync53/1 -> Out53/1

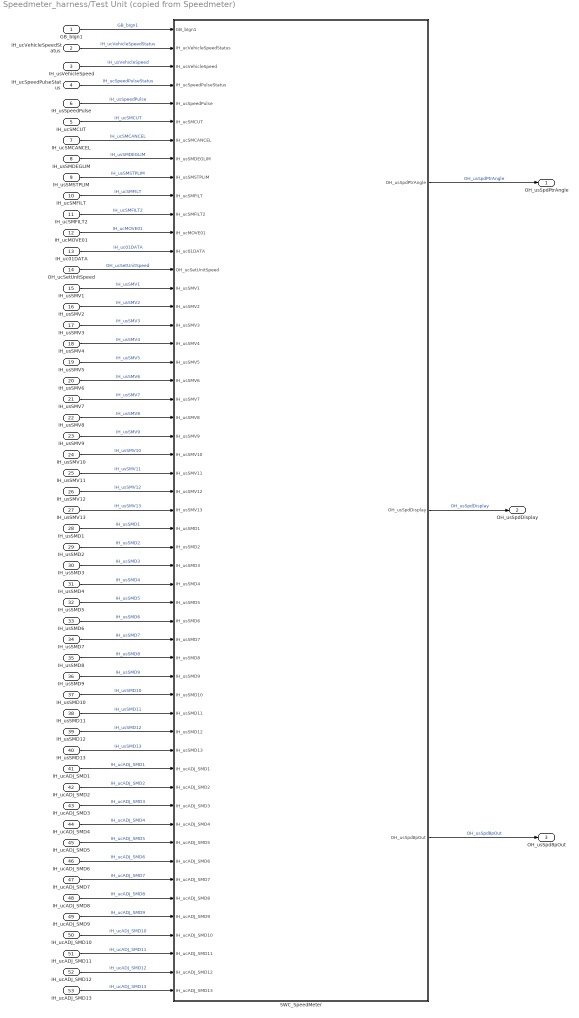
== system Speedmeter_harness/Test Unit (copied from Speedmeter) ==
  GB_bIgn1 : Inport  OutMin=0  OutMax=1  OutDataTypeStr=uint8  SampleTime=STEP_TIME
  IH_ucVehicleSpeedStatus : Inport  Port=2  OutMin=0  OutMax=3  OutDataTypeStr=fixdt(0,8,1,0)  SampleTime=STEP_TIME
  IH_usVehicleSpeed : Inport  Port=3  OutMin=0  OutMax=655.35  OutDataTypeStr=fixdt(0,16,0.01,0)  SampleTime=STEP_TIME
  IH_ucSpeedPulseStatus : Inport  Port=4  OutMin=0  OutMax=3  OutDataTypeStr=fixdt(0,8,1,0)  SampleTime=STEP_TIME
  IH_ucSMCUT : Inport  Port=5  OutMin=0  OutMax=3  OutDataTypeStr=fixdt(0,8,1,0)  SampleTime=STEP_TIME
  IH_usSpeedPulse : Inport  Port=6  OutMin=0  OutMax=655.35  OutDataTypeStr=fixdt(0,16,0.01,0)  SampleTime=STEP_TIME
  IH_ucSMCANCEL : Inport  Port=7  OutMin=0  OutMax=10.8996  OutDataTypeStr=fixdt(0,8,0.3516,0)  SampleTime=STEP_TIME
  IH_usSMDEGLIM : Inport  Port=8  OutMin=0  OutMax=359.6868  OutDataTypeStr=fixdt(0,16,0.3516,0)  SampleTime=STEP_TIME
  IH_usSMSTPLIM : Inport  Port=9  OutMin=0  OutMax=5.5377  OutDataTypeStr=fixdt(0,16,0.0879,0)  SampleTime=STEP_TIME
  IH_ucSMFILT : Inport  Port=10  OutMin=0  OutMax=7  OutDataTypeStr=fixdt(0,8,1,0)  SampleTime=STEP_TIME
  IH_ucSMFILT2 : Inport  Port=11  OutMin=0  OutMax=7  OutDataTypeStr=fixdt(0,8,1,0)  SampleTime=STEP_TIME
  IH_ucMOVE01 : Inport  Port=12  OutMin=0  OutMax=3  OutDataTypeStr=fixdt(0,8,1,0)  SampleTime=STEP_TIME
  IH_uc01DATA : Inport  Port=13  OutMin=0  OutMax=1  OutDataTypeStr=fixdt(0,8,1,0)  SampleTime=STEP_TIME
  OH_ucSetUnitSpeed : Inport  Port=14  OutMin=0  OutMax=1  OutDataTypeStr=fixdt(0,8,1,0)  SampleTime=STEP_TIME
  IH_usSMV1 : Inport  Port=15  OutMin=0  OutMax=409.5  OutDataTypeStr=fixdt(0,16,0.1,0)  SampleTime=STEP_TIME
  IH_usSMV2 : Inport  Port=16  OutMin=0  OutMax=409.5  OutDataTypeStr=fixdt(0,16,0.1,0)  SampleTime=STEP_TIME
  IH_usSMV3 : Inport  Port=17  OutMin=0  OutMax=409.5  OutDataTypeStr=fixdt(0,16,0.1,0)  SampleTime=STEP_TIME
  IH_usSMV4 : Inport  Port=18  OutMin=0  OutMax=409.5  OutDataTypeStr=fixdt(0,16,0.1,0)  SampleTime=STEP_TIME
  IH_usSMV5 : Inport  Port=19  OutMin=0  OutMax=409.5  OutDataTypeStr=fixdt(0,16,0.1,0)  SampleTime=STEP_TIME
  IH_usSMV6 : Inport  Port=20  OutMin=0  OutMax=409.5  OutDataTypeStr=fixdt(0,16,0.1,0)  SampleTime=STEP_TIME
  IH_usSMV7 : Inport  Port=21  OutMin=0  OutMax=409.5  OutDataTypeStr=fixdt(0,16,0.1,0)  SampleTime=STEP_TIME
  IH_usSMV8 : Inport  Port=22  OutMin=0  OutMax=409.5  OutDataTypeStr=fixdt(0,16,0.1,0)  SampleTime=STEP_TIME
  IH_usSMV9 : Inport  Port=23  OutMin=0  OutMax=409.5  OutDataTypeStr=fixdt(0,16,0.1,0)  SampleTime=STEP_TIME
  IH_usSMV10 : Inport  Port=24  OutMin=0  OutMax=409.5  OutDataTypeStr=fixdt(0,16,0.1,0)  SampleTime=STEP_TIME
  IH_usSMV11 : Inport  Port=25  OutMin=0  OutMax=409.5  OutDataTypeStr=fixdt(0,16,0.1,0)  SampleTime=STEP_TIME
  IH_usSMV12 : Inport  Port=26  OutMin=0  OutMax=409.5  OutDataTypeStr=fixdt(0,16,0.1,0)  SampleTime=STEP_TIME
  IH_usSMV13 : Inport  Port=27  OutMin=0  OutMax=409.5  OutDataTypeStr=fixdt(0,16,0.1,0)  SampleTime=STEP_TIME
  IH_usSMD1 : Inport  Port=28  OutMin=0  OutMax=359.9505  OutDataTypeStr=fixdt(0,16,0.0879,0)  SampleTime=STEP_TIME
  IH_usSMD2 : Inport  Port=29  OutMin=0  OutMax=359.9505  OutDataTypeStr=fixdt(0,16,0.0879,0)  SampleTime=STEP_TIME
  IH_usSMD3 : Inport  Port=30  OutMin=0  OutMax=359.9505  OutDataTypeStr=fixdt(0,16,0.0879,0)  SampleTime=STEP_TIME
  IH_usSMD4 : Inport  Port=31  OutMin=0  OutMax=359.9505  OutDataTypeStr=fixdt(0,16,0.0879,0)  SampleTime=STEP_TIME
  IH_usSMD5 : Inport  Port=32  OutMin=0  OutMax=359.9505  OutDataTypeStr=fixdt(0,16,0.0879,0)  SampleTime=STEP_TIME
  IH_usSMD6 : Inport  Port=33  OutMin=0  OutMax=359.9505  OutDataTypeStr=fixdt(0,16,0.0879,0)  SampleTime=STEP_TIME
  IH_usSMD7 : Inport  Port=34  OutMin=0  OutMax=359.9505  OutDataTypeStr=fixdt(0,16,0.0879,0)  SampleTime=STEP_TIME
  IH_usSMD8 : Inport  Port=35  OutMin=0  OutMax=359.9505  OutDataTypeStr=fixdt(0,16,0.0879,0)  SampleTime=STEP_TIME
  IH_usSMD9 : Inport  Port=36  OutMin=0  OutMax=359.9505  OutDataTypeStr=fixdt(0,16,0.0879,0)  SampleTime=STEP_TIME
  IH_usSMD10 : Inport  Port=37  OutMin=0  OutMax=359.9505  OutDataTypeStr=fixdt(0,16,0.0879,0)  SampleTime=STEP_TIME
  IH_usSMD11 : Inport  Port=38  OutMin=0  OutMax=359.9505  OutDataTypeStr=fixdt(0,16,0.0879,0)  SampleTime=STEP_TIME
  IH_usSMD12 : Inport  Port=39  OutMin=0  OutMax=359.9505  OutDataTypeStr=fixdt(0,16,0.0879,0)  SampleTime=STEP_TIME
  IH_usSMD13 : Inport  Port=40  OutMin=0  OutMax=359.9505  OutDataTypeStr=fixdt(0,16,0.0879,0)  SampleTime=STEP_TIME
  IH_ucADJ_SMD1 : Inport  Port=41  OutMin=0  OutMax=22.4145  OutDataTypeStr=fixdt(0,8,0.0879,0)  SampleTime=STEP_TIME
  IH_ucADJ_SMD2 : Inport  Port=42  OutMin=0  OutMax=22.4145  OutDataTypeStr=fixdt(0,8,0.0879,0)  SampleTime=STEP_TIME
  IH_ucADJ_SMD3 : Inport  Port=43  OutMin=0  OutMax=22.4145  OutDataTypeStr=fixdt(0,8,0.0879,0)  SampleTime=STEP_TIME
  IH_ucADJ_SMD4 : Inport  Port=44  OutMin=0  OutMax=22.4145  OutDataTypeStr=fixdt(0,8,0.0879,0)  SampleTime=STEP_TIME
  IH_ucADJ_SMD5 : Inport  Port=45  OutMin=0  OutMax=22.4145  OutDataTypeStr=fixdt(0,8,0.0879,0)  SampleTime=STEP_TIME
  IH_ucADJ_SMD6 : Inport  Port=46  OutMin=0  OutMax=22.4145  OutDataTypeStr=fixdt(0,8,0.0879,0)  SampleTime=STEP_TIME
  IH_ucADJ_SMD7 : Inport  Port=47  OutMin=0  OutMax=22.4145  OutDataTypeStr=fixdt(0,8,0.0879,0)  SampleTime=STEP_TIME
  IH_ucADJ_SMD8 : Inport  Port=48  OutMin=0  OutMax=22.4145  OutDataTypeStr=fixdt(0,8,0.0879,0)  SampleTime=STEP_TIME
  IH_ucADJ_SMD9 : Inport  Port=49  OutMin=0  OutMax=22.4145  OutDataTypeStr=fixdt(0,8,0.0879,0)  SampleTime=STEP_TIME
  IH_ucADJ_SMD10 : Inport  Port=50  OutMin=0  OutMax=22.4145  OutDataTypeStr=fixdt(0,8,0.0879,0)  SampleTime=STEP_TIME
  IH_ucADJ_SMD11 : Inport  Port=51  OutMin=0  OutMax=22.4145  OutDataTypeStr=fixdt(0,8,0.0879,0)  SampleTime=STEP_TIME
  IH_ucADJ_SMD12 : Inport  Port=52  OutMin=0  OutMax=22.4145  OutDataTypeStr=fixdt(0,8,0.0879,0)  SampleTime=STEP_TIME
  IH_ucADJ_SMD13 : Inport  Port=53  OutMin=0  OutMax=22.4145  OutDataTypeStr=fixdt(0,8,0.0879,0)  SampleTime=STEP_TIME
  SWC_SpeedMeter : Subsystem  LoadFcn=set_param('Speedmeter', 'DataTypeOverride','Single')  TreatAsAtomicUnit=on
  OH_usSpdPtrAngle : Outport  OutMin=0  OutMax=4095  OutDataTypeStr=fixdt(0,16,0.0879,0)  SampleTime=STEP_TIME  VectorParamsAs1DForOutWhenUnconnected=off
  OH_usSpdDisplay : Outport  Port=2  OutDataTypeStr=fixdt(0,16,1,0)  SampleTime=STEP_TIME  VectorParamsAs1DForOutWhenUnconnected=off
  OH_usSpd8pOut : Outport  Port=3  OutMin=0  OutMax=655.34  OutDataTypeStr=fixdt(0,16,0.01,0)  SampleTime=STEP_TIME  VectorParamsAs1DForOutWhenUnconnected=off
  wires:
  IH_ucVehicleSpeedStatus/1 -> SWC_SpeedMeter/2(IH_ucVehicleSpeedStatus)  "IH_ucVehicleSpeedStatus"
  IH_usSMV12/1 -> SWC_SpeedMeter/26(IH_usSMV12)  "IH_usSMV12"
  GB_bIgn1/1 -> SWC_SpeedMeter/1(GB_bIgn1)  "GB_bIgn1"
  IH_ucADJ_SMD6/1 -> SWC_SpeedMeter/46(IH_ucADJ_SMD6)  "IH_ucADJ_SMD6"
  IH_ucADJ_SMD7/1 -> SWC_SpeedMeter/47(IH_ucADJ_SMD7)  "IH_ucADJ_SMD7"
  IH_uc01DATA/1 -> SWC_SpeedMeter/13(IH_uc01DATA)  "IH_uc01DATA"
  IH_ucADJ_SMD12/1 -> SWC_SpeedMeter/52(IH_ucADJ_SMD12)  "IH_ucADJ_SMD12"
  IH_ucADJ_SMD13/1 -> SWC_SpeedMeter/53(IH_ucADJ_SMD13)  "IH_ucADJ_SMD13"
  IH_usVehicleSpeed/1 -> SWC_SpeedMeter/3(IH_usVehicleSpeed)  "IH_usVehicleSpeed"
  IH_ucADJ_SMD11/1 -> SWC_SpeedMeter/51(IH_ucADJ_SMD11)  "IH_ucADJ_SMD11"
  IH_ucADJ_SMD8/1 -> SWC_SpeedMeter/48(IH_ucADJ_SMD8)  "IH_ucADJ_SMD8"
  IH_usSMD9/1 -> SWC_SpeedMeter/36(IH_usSMD9)  "IH_usSMD9"
  IH_usSMD11/1 -> SWC_SpeedMeter/38(IH_usSMD11)  "IH_usSMD11"
  IH_usSMV2/1 -> SWC_SpeedMeter/16(IH_usSMV2)  "IH_usSMV2"
  IH_ucADJ_SMD3/1 -> SWC_SpeedMeter/43(IH_ucADJ_SMD3)  "IH_ucADJ_SMD3"
  IH_usSMD10/1 -> SWC_SpeedMeter/37(IH_usSMD10)  "IH_usSMD10"
  IH_usSMD3/1 -> SWC_SpeedMeter/30(IH_usSMD3)  "IH_usSMD3"
  IH_usSMD13/1 -> SWC_SpeedMeter/40(IH_usSMD13)  "IH_usSMD13"
  OH_ucSetUnitSpeed/1 -> SWC_SpeedMeter/14(OH_ucSetUnitSpeed)  "OH_ucSetUnitSpeed"
  IH_usSMDEGLIM/1 -> SWC_SpeedMeter/8(IH_usSMDEGLIM)  "IH_usSMDEGLIM"
  IH_usSMV13/1 -> SWC_SpeedMeter/27(IH_usSMV13)  "IH_usSMV13"
  IH_usSpeedPulse/1 -> SWC_SpeedMeter/5(IH_usSpeedPulse)  "IH_usSpeedPulse"
  IH_ucADJ_SMD5/1 -> SWC_SpeedMeter/45(IH_ucADJ_SMD5)  "IH_ucADJ_SMD5"
  IH_usSMD5/1 -> SWC_SpeedMeter/32(IH_usSMD5)  "IH_usSMD5"
  IH_ucSMCUT/1 -> SWC_SpeedMeter/6(IH_ucSMCUT)  "IH_ucSMCUT"
  IH_ucSMFILT2/1 -> SWC_SpeedMeter/11(IH_ucSMFILT2)  "IH_ucSMFILT2"
  IH_ucADJ_SMD2/1 -> SWC_SpeedMeter/42(IH_ucADJ_SMD2)  "IH_ucADJ_SMD2"
  IH_usSMD2/1 -> SWC_SpeedMeter/29(IH_usSMD2)  "IH_usSMD2"
  IH_usSMV9/1 -> SWC_SpeedMeter/23(IH_usSMV9)  "IH_usSMV9"
  IH_usSMV8/1 -> SWC_SpeedMeter/22(IH_usSMV8)  "IH_usSMV8"
  IH_usSMD4/1 -> SWC_SpeedMeter/31(IH_usSMD4)  "IH_usSMD4"
  IH_ucSpeedPulseStatus/1 -> SWC_SpeedMeter/4(IH_ucSpeedPulseStatus)  "IH_ucSpeedPulseStatus"
  IH_usSMD6/1 -> SWC_SpeedMeter/33(IH_usSMD6)  "IH_usSMD6"
  IH_usSMV7/1 -> SWC_SpeedMeter/21(IH_usSMV7)  "IH_usSMV7"
  IH_ucADJ_SMD4/1 -> SWC_SpeedMeter/44(IH_ucADJ_SMD4)  "IH_ucADJ_SMD4"
  IH_usSMSTPLIM/1 -> SWC_SpeedMeter/9(IH_usSMSTPLIM)  "IH_usSMSTPLIM"
  IH_usSMD8/1 -> SWC_SpeedMeter/35(IH_usSMD8)  "IH_usSMD8"
  IH_ucADJ_SMD9/1 -> SWC_SpeedMeter/49(IH_ucADJ_SMD9)  "IH_ucADJ_SMD9"
  IH_usSMV5/1 -> SWC_SpeedMeter/19(IH_usSMV5)  "IH_usSMV5"
  IH_usSMD12/1 -> SWC_SpeedMeter/39(IH_usSMD12)  "IH_usSMD12"
  IH_ucSMFILT/1 -> SWC_SpeedMeter/10(IH_ucSMFILT)  "IH_ucSMFILT"
  IH_usSMD1/1 -> SWC_SpeedMeter/28(IH_usSMD1)  "IH_usSMD1"
  IH_usSMV10/1 -> SWC_SpeedMeter/24(IH_usSMV10)  "IH_usSMV10"
  IH_usSMV3/1 -> SWC_SpeedMeter/17(IH_usSMV3)  "IH_usSMV3"
  IH_ucMOVE01/1 -> SWC_SpeedMeter/12(IH_ucMOVE01)  "IH_ucMOVE01"
  IH_ucADJ_SMD10/1 -> SWC_SpeedMeter/50(IH_ucADJ_SMD10)  "IH_ucADJ_SMD10"
  IH_usSMV1/1 -> SWC_SpeedMeter/15(IH_usSMV1)  "IH_usSMV1"
  IH_usSMV4/1 -> SWC_SpeedMeter/18(IH_usSMV4)  "IH_usSMV4"
  IH_usSMV6/1 -> SWC_SpeedMeter/20(IH_usSMV6)  "IH_usSMV6"
  IH_usSMV11/1 -> SWC_SpeedMeter/25(IH_usSMV11)  "IH_usSMV11"
  IH_ucADJ_SMD1/1 -> SWC_SpeedMeter/41(IH_ucADJ_SMD1)  "IH_ucADJ_SMD1"
  IH_ucSMCANCEL/1 -> SWC_SpeedMeter/7(IH_ucSMCANCEL)  "IH_ucSMCANCEL"
  IH_usSMD7/1 -> SWC_SpeedMeter/34(IH_usSMD7)  "IH_usSMD7"
  SWC_SpeedMeter/3(OH_usSpd8pOut) -> OH_usSpd8pOut/1  "OH_usSpd8pOut"
  SWC_SpeedMeter/1(OH_usSpdPtrAngle) -> OH_usSpdPtrAngle/1  "OH_usSpdPtrAngle"
  SWC_SpeedMeter/2(OH_usSpdDisplay) -> OH_usSpdDisplay/1  "OH_usSpdDisplay"

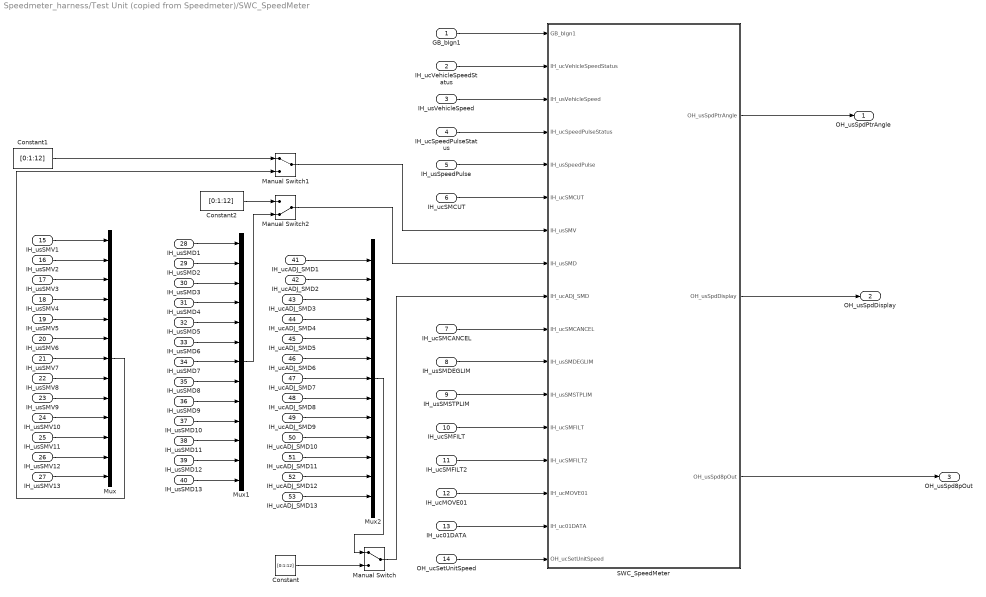
== system Speedmeter_harness/Test Unit (copied from Speedmeter)/SWC_SpeedMeter ==
  GB_bIgn1 : Inport  SampleTime=STEP_TIME
  IH_ucVehicleSpeedStatus : Inport  Port=2  OutDataTypeStr=fixdt(0,8,1,0)  SampleTime=STEP_TIME
  IH_usVehicleSpeed : Inport  Port=3  OutDataTypeStr=fixdt(0,16,0.01,0)  SampleTime=STEP_TIME
  IH_ucSpeedPulseStatus : Inport  Port=4  OutDataTypeStr=fixdt(0,8,1,0)  SampleTime=STEP_TIME
  IH_usSpeedPulse : Inport  Port=5  OutDataTypeStr=fixdt(0,16,0.01,0)  SampleTime=STEP_TIME
  IH_ucSMCUT : Inport  Port=6  OutDataTypeStr=fixdt(0,8,1,0)  SampleTime=STEP_TIME
  IH_ucSMCANCEL : Inport  Port=7  SampleTime=STEP_TIME
  IH_usSMDEGLIM : Inport  Port=8  SampleTime=STEP_TIME
  IH_usSMSTPLIM : Inport  Port=9  SampleTime=STEP_TIME
  IH_ucSMFILT : Inport  Port=10  OutDataTypeStr=fixdt(0,8,1,0)  SampleTime=STEP_TIME
  IH_ucSMFILT2 : Inport  Port=11  OutDataTypeStr=fixdt(0,8,1,0)  SampleTime=STEP_TIME
  IH_ucMOVE01 : Inport  Port=12  OutDataTypeStr=fixdt(0,8,1,0)  SampleTime=STEP_TIME
  IH_uc01DATA : Inport  Port=13  OutDataTypeStr=fixdt(0,8,1,0)  SampleTime=STEP_TIME
  OH_ucSetUnitSpeed : Inport  Port=14  OutDataTypeStr=fixdt(0,8,1,0)  SampleTime=STEP_TIME
  IH_usSMV1 : Inport  Port=15  SampleTime=STEP_TIME
  IH_usSMV2 : Inport  Port=16  SampleTime=STEP_TIME
  IH_usSMV3 : Inport  Port=17  SampleTime=STEP_TIME
  IH_usSMV4 : Inport  Port=18  SampleTime=STEP_TIME
  IH_usSMV5 : Inport  Port=19  SampleTime=STEP_TIME
  IH_usSMV6 : Inport  Port=20  SampleTime=STEP_TIME
  IH_usSMV7 : Inport  Port=21  SampleTime=STEP_TIME
  IH_usSMV8 : Inport  Port=22  SampleTime=STEP_TIME
  IH_usSMV9 : Inport  Port=23  SampleTime=STEP_TIME
  IH_usSMV10 : Inport  Port=24  SampleTime=STEP_TIME
  IH_usSMV11 : Inport  Port=25  SampleTime=STEP_TIME
  IH_usSMV12 : Inport  Port=26  SampleTime=STEP_TIME
  IH_usSMV13 : Inport  Port=27  SampleTime=STEP_TIME
  IH_usSMD1 : Inport  Port=28  SampleTime=STEP_TIME
  IH_usSMD2 : Inport  Port=29  SampleTime=STEP_TIME
  IH_usSMD3 : Inport  Port=30  SampleTime=STEP_TIME
  IH_usSMD4 : Inport  Port=31  SampleTime=STEP_TIME
  IH_usSMD5 : Inport  Port=32  SampleTime=STEP_TIME
  IH_usSMD6 : Inport  Port=33  SampleTime=STEP_TIME
  IH_usSMD7 : Inport  Port=34  SampleTime=STEP_TIME
  IH_usSMD8 : Inport  Port=35  SampleTime=STEP_TIME
  IH_usSMD9 : Inport  Port=36  SampleTime=STEP_TIME
  IH_usSMD10 : Inport  Port=37  SampleTime=STEP_TIME
  IH_usSMD11 : Inport  Port=38  SampleTime=STEP_TIME
  IH_usSMD12 : Inport  Port=39  SampleTime=STEP_TIME
  IH_usSMD13 : Inport  Port=40  SampleTime=STEP_TIME
  IH_ucADJ_SMD1 : Inport  Port=41  SampleTime=STEP_TIME
  IH_ucADJ_SMD2 : Inport  Port=42  SampleTime=STEP_TIME
  IH_ucADJ_SMD3 : Inport  Port=43  SampleTime=STEP_TIME
  IH_ucADJ_SMD4 : Inport  Port=44  SampleTime=STEP_TIME
  IH_ucADJ_SMD5 : Inport  Port=45  SampleTime=STEP_TIME
  IH_ucADJ_SMD6 : Inport  Port=46  SampleTime=STEP_TIME
  IH_ucADJ_SMD7 : Inport  Port=47  SampleTime=STEP_TIME
  IH_ucADJ_SMD8 : Inport  Port=48  SampleTime=STEP_TIME
  IH_ucADJ_SMD9 : Inport  Port=49  SampleTime=STEP_TIME
  IH_ucADJ_SMD10 : Inport  Port=50  SampleTime=STEP_TIME
  IH_ucADJ_SMD11 : Inport  Port=51  SampleTime=STEP_TIME
  IH_ucADJ_SMD12 : Inport  Port=52  SampleTime=STEP_TIME
  IH_ucADJ_SMD13 : Inport  Port=53  SampleTime=STEP_TIME
  Constant : Constant  Value=[0:1:12]  OutDataTypeStr=fixdt(0,8,0.0879,0)
  Constant1 : Constant  Value=[0:1:12]  OutDataTypeStr=fixdt(0,16,0.1,0)
  Constant2 : Constant  Value=[0:1:12]  OutDataTypeStr=fixdt(0,16,0.0879,0)
  Manual Switch : ManualSwitch
  Manual Switch1 : ManualSwitch
  Manual Switch2 : ManualSwitch  CurrentSetting=0
  Mux : Mux  Inputs=13
  Mux1 : Mux  Inputs=13
  Mux2 : Mux  Inputs=13
  SWC_SpeedMeter : Subsystem  TreatAsAtomicUnit=on
  OH_usSpdPtrAngle : Outport  OutMin=0  OutMax=4095  OutDataTypeStr=fixdt(0,16,0.0879,0)  SampleTime=STEP_TIME  VectorParamsAs1DForOutWhenUnconnected=off
  OH_usSpdDisplay : Outport  Port=2  SampleTime=STEP_TIME  VectorParamsAs1DForOutWhenUnconnected=off
  OH_usSpd8pOut : Outport  Port=3  OutMin=0  OutMax=655.34  OutDataTypeStr=fixdt(0,16,0.01,0)  SampleTime=STEP_TIME  VectorParamsAs1DForOutWhenUnconnected=off
  wires:
  IH_uc01DATA/1 -> SWC_SpeedMeter/16(IH_uc01DATA)
  IH_ucMOVE01/1 -> SWC_SpeedMeter/15(IH_ucMOVE01)
  IH_ucSpeedPulseStatus/1 -> SWC_SpeedMeter/4(IH_ucSpeedPulseStatus)
  IH_ucVehicleSpeedStatus/1 -> SWC_SpeedMeter/2(IH_ucVehicleSpeedStatus)
  GB_bIgn1/1 -> SWC_SpeedMeter/1(GB_bIgn1)
  IH_usSMD3/1 -> Mux1/3
  IH_usSMD10/1 -> Mux1/10
  IH_usSMD13/1 -> Mux1/13
  IH_usSMD4/1 -> Mux1/4
  IH_usSMV9/1 -> Mux/9
  IH_usSMD5/1 -> Mux1/5
  IH_usSMV1/1 -> Mux/1
  IH_usSMV8/1 -> Mux/8
  IH_usSMV7/1 -> Mux/7
  IH_usSMV5/1 -> Mux/5
  IH_usSMV10/1 -> Mux/10
  IH_usSMV13/1 -> Mux/13
  Mux/1 -> Manual Switch1/2
  Constant2/1 -> Manual Switch2/1
  Manual Switch1/1 -> SWC_SpeedMeter/7(IH_usSMV)
  SWC_SpeedMeter/1(OH_usSpdPtrAngle) -> OH_usSpdPtrAngle/1
  IH_usSMD8/1 -> Mux1/8
  OH_ucSetUnitSpeed/1 -> SWC_SpeedMeter/17(OH_ucSetUnitSpeed)
  IH_usSMSTPLIM/1 -> SWC_SpeedMeter/12(IH_usSMSTPLIM)
  SWC_SpeedMeter/3(OH_usSpd8pOut) -> OH_usSpd8pOut/1
  IH_usSMD2/1 -> Mux1/2
  IH_ucSMFILT2/1 -> SWC_SpeedMeter/14(IH_ucSMFILT2)
  IH_usSMV6/1 -> Mux/6
  IH_usSMV4/1 -> Mux/4
  IH_usSMDEGLIM/1 -> SWC_SpeedMeter/11(IH_usSMDEGLIM)
  SWC_SpeedMeter/2(OH_usSpdDisplay) -> OH_usSpdDisplay/1
  IH_ucSMCANCEL/1 -> SWC_SpeedMeter/10(IH_ucSMCANCEL)
  IH_usSpeedPulse/1 -> SWC_SpeedMeter/5(IH_usSpeedPulse)
  IH_usSMD9/1 -> Mux1/9
  IH_usSMD7/1 -> Mux1/7
  IH_ucADJ_SMD9/1 -> Mux2/9
  IH_usVehicleSpeed/1 -> SWC_SpeedMeter/3(IH_usVehicleSpeed)
  IH_usSMV2/1 -> Mux/2
  IH_ucSMFILT/1 -> SWC_SpeedMeter/13(IH_ucSMFILT)
  IH_ucADJ_SMD12/1 -> Mux2/12
  Constant/1 -> Manual Switch/2
  IH_ucADJ_SMD6/1 -> Mux2/6
  IH_ucADJ_SMD1/1 -> Mux2/1
  Mux2/1 -> Manual Switch/1
  IH_ucADJ_SMD13/1 -> Mux2/13
  IH_ucSMCUT/1 -> SWC_SpeedMeter/6(IH_ucSMCUT)
  IH_ucADJ_SMD5/1 -> Mux2/5
  IH_usSMD12/1 -> Mux1/12
  IH_usSMD1/1 -> Mux1/1
  IH_ucADJ_SMD11/1 -> Mux2/11
  IH_ucADJ_SMD8/1 -> Mux2/8
  Manual Switch2/1 -> SWC_SpeedMeter/8(IH_usSMD)
  IH_usSMD11/1 -> Mux1/11
  Manual Switch/1 -> SWC_SpeedMeter/9(IH_ucADJ_SMD)
  IH_usSMD6/1 -> Mux1/6
  IH_usSMV3/1 -> Mux/3
  IH_usSMV12/1 -> Mux/12
  IH_ucADJ_SMD7/1 -> Mux2/7
  IH_ucADJ_SMD2/1 -> Mux2/2
  IH_usSMV11/1 -> Mux/11
  Constant1/1 -> Manual Switch1/1
  IH_ucADJ_SMD10/1 -> Mux2/10
  IH_ucADJ_SMD4/1 -> Mux2/4
  Mux1/1 -> Manual Switch2/2
  IH_ucADJ_SMD3/1 -> Mux2/3

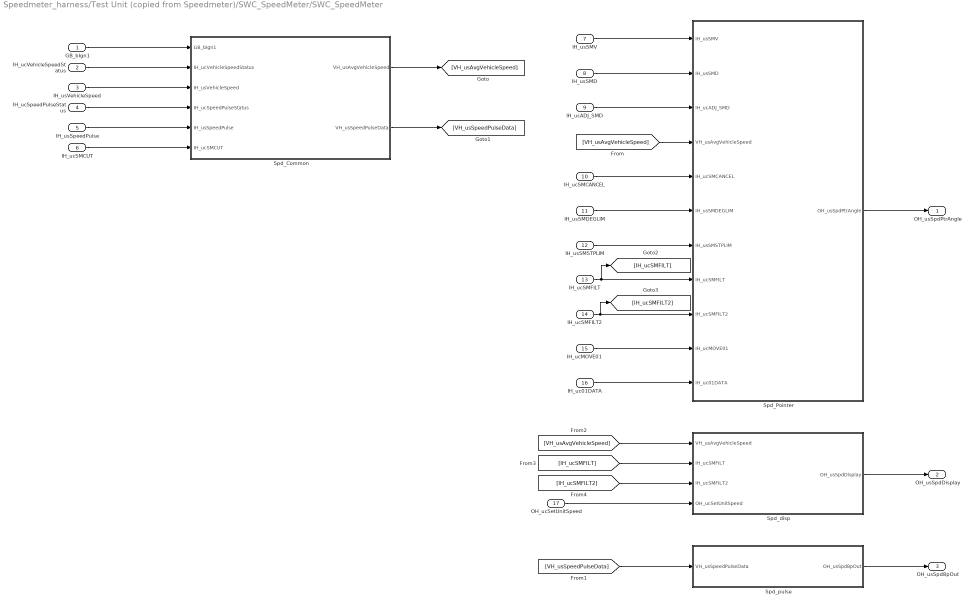
== system Speedmeter_harness/Test Unit (copied from Speedmeter)/SWC_SpeedMeter/SWC_SpeedMeter ==
  GB_bIgn1 : Inport  SampleTime=STEP_TIME
  IH_ucVehicleSpeedStatus : Inport  Port=2  OutDataTypeStr=fixdt(0,8,1,0)  SampleTime=STEP_TIME
  IH_usVehicleSpeed : Inport  Port=3  OutDataTypeStr=fixdt(0,16,0.01,0)  SampleTime=STEP_TIME
  IH_ucSpeedPulseStatus : Inport  Port=4  OutDataTypeStr=fixdt(0,8,1,0)  SampleTime=STEP_TIME
  IH_usSpeedPulse : Inport  Port=5  OutDataTypeStr=fixdt(0,16,0.01,0)  SampleTime=STEP_TIME
  IH_ucSMCUT : Inport  Port=6  OutDataTypeStr=fixdt(0,8,1,0)  SampleTime=STEP_TIME
  IH_usSMV : Inport  Port=7  SampleTime=STEP_TIME
  IH_usSMD : Inport  Port=8  SampleTime=STEP_TIME
  IH_ucADJ_SMD : Inport  Port=9  SampleTime=STEP_TIME
  IH_ucSMCANCEL : Inport  Port=10  SampleTime=STEP_TIME
  IH_usSMDEGLIM : Inport  Port=11  SampleTime=STEP_TIME
  IH_usSMSTPLIM : Inport  Port=12  SampleTime=STEP_TIME
  IH_ucSMFILT : Inport  Port=13  OutDataTypeStr=fixdt(0,8,1,0)  SampleTime=STEP_TIME
  IH_ucSMFILT2 : Inport  Port=14  OutDataTypeStr=fixdt(0,8,1,0)  SampleTime=STEP_TIME
  IH_ucMOVE01 : Inport  Port=15  OutDataTypeStr=fixdt(0,8,1,0)  SampleTime=STEP_TIME
  IH_uc01DATA : Inport  Port=16  OutDataTypeStr=fixdt(0,8,1,0)  SampleTime=STEP_TIME
  OH_ucSetUnitSpeed : Inport  Port=17  OutDataTypeStr=fixdt(0,8,1,0)  SampleTime=STEP_TIME
  Spd_Common : Subsystem  TreatAsAtomicUnit=on
  Spd_Pointer : Subsystem  TreatAsAtomicUnit=on
  Spd_disp : Subsystem  TreatAsAtomicUnit=on
  Spd_pulse : Subsystem  TreatAsAtomicUnit=on
  OH_usSpdPtrAngle : Outport  SampleTime=STEP_TIME  VectorParamsAs1DForOutWhenUnconnected=off
  OH_usSpdDisplay : Outport  Port=2  SampleTime=STEP_TIME  VectorParamsAs1DForOutWhenUnconnected=off
  OH_usSpd8pOut : Outport  Port=3  OutMin=0  OutMax=655.34  OutDataTypeStr=fixdt(0,16,0.01,0)  SampleTime=STEP_TIME  VectorParamsAs1DForOutWhenUnconnected=off
  wires:
  IH_uc01DATA/1 -> Spd_Pointer/11(IH_uc01DATA)
  IH_ucMOVE01/1 -> Spd_Pointer/10(IH_ucMOVE01)
  IH_ucSpeedPulseStatus/1 -> Spd_Common/4(IH_ucSpeedPulseStatus)
  IH_ucVehicleSpeedStatus/1 -> Spd_Common/2(IH_ucVehicleSpeedStatus)
  GB_bIgn1/1 -> Spd_Common/1(GB_bIgn1)
  IH_ucSMFILT/1 -> [IH_ucSMFILT], Spd_Pointer/8(IH_ucSMFILT)
  [IH_ucSMFILT2] -> Spd_disp/3(IH_ucSMFILT2)
  Spd_disp/1(OH_usSpdDisplay) -> OH_usSpdDisplay/1
  [IH_ucSMFILT] -> Spd_disp/2(IH_ucSMFILT)
  IH_ucSMCANCEL/1 -> Spd_Pointer/5(IH_ucSMCANCEL)
  IH_usSMDEGLIM/1 -> Spd_Pointer/6(IH_usSMDEGLIM)
  [VH_usSpeedPulseData] -> Spd_pulse/1(VH_usSpeedPulseData)
  Spd_Pointer/1(OH_usSpdPtrAngle) -> OH_usSpdPtrAngle/1
  IH_ucADJ_SMD/1 -> Spd_Pointer/3(IH_ucADJ_SMD)
  OH_ucSetUnitSpeed/1 -> Spd_disp/4(OH_ucSetUnitSpeed)
  IH_usSMSTPLIM/1 -> Spd_Pointer/7(IH_usSMSTPLIM)
  [VH_usAvgVehicleSpeed] -> Spd_Pointer/4(VH_usAvgVehicleSpeed)
  IH_usSMV/1 -> Spd_Pointer/1(IH_usSMV)
  IH_ucSMFILT2/1 -> Spd_Pointer/9(IH_ucSMFILT2), [IH_ucSMFILT2]
  Spd_pulse/1(OH_usSpd8pOut) -> OH_usSpd8pOut/1
  [VH_usAvgVehicleSpeed] -> Spd_disp/1(VH_usAvgVehicleSpeed)
  IH_usSMD/1 -> Spd_Pointer/2(IH_usSMD)
  Spd_Common/1(VH_usAvgVehicleSpeed) -> [VH_usAvgVehicleSpeed]
  IH_usSpeedPulse/1 -> Spd_Common/5(IH_usSpeedPulse)
  IH_usVehicleSpeed/1 -> Spd_Common/3(IH_usVehicleSpeed)
  Spd_Common/2(VH_usSpeedPulseData) -> [VH_usSpeedPulseData]
  IH_ucSMCUT/1 -> Spd_Common/6(IH_ucSMCUT)

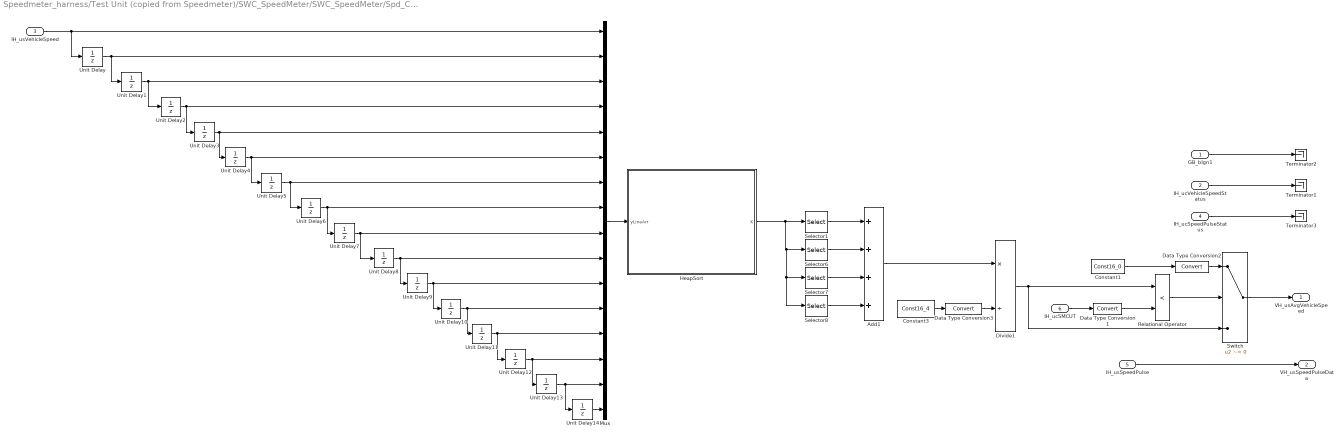
== system Speedmeter_harness/Test Unit (copied from Speedmeter)/SWC_SpeedMeter/SWC_SpeedMeter/Spd_Common ==
  GB_bIgn1 : Inport  SampleTime=STEP_TIME
  IH_ucVehicleSpeedStatus : Inport  Port=2  OutDataTypeStr=fixdt(0,8,1,0)  SampleTime=STEP_TIME
  IH_usVehicleSpeed : Inport  Port=3  OutDataTypeStr=fixdt(0,16,0.01,0)  SampleTime=STEP_TIME
  IH_ucSpeedPulseStatus : Inport  Port=4  OutDataTypeStr=fixdt(0,8,1,0)  SampleTime=STEP_TIME
  IH_usSpeedPulse : Inport  Port=5  OutDataTypeStr=fixdt(0,16,0.01,0)  SampleTime=STEP_TIME
  IH_ucSMCUT : Inport  Port=6  OutDataTypeStr=fixdt(0,8,1,0)  SampleTime=STEP_TIME
  Add1 : Sum  Inputs=++++  OutDataTypeStr=fixdt(0,32,0.01,0)  InputSameDT=on
  Constant1 : Constant  Value=Const16_0  SampleTime=STEP_TIME
  Constant3 : Constant  Value=Const16_4  OutDataTypeStr=uint16  SampleTime=STEP_TIME
  Data Type Conversion1 : DataTypeConversion
  Data Type Conversion2 : DataTypeConversion
  Data Type Conversion3 : DataTypeConversion
  Divide1 : Product  Inputs=*/  OutDataTypeStr=Inherit: Inherit via back propagation  InputSameDT=on
  HeapSort : Stateflow chart  TreatAsAtomicUnit=on
  Mux : Mux  Inputs=16
  Relational Operator : RelationalOperator  Operator=<  OutDataTypeStr=boolean  RndMeth=Simplest  InputSameDT=on
  Selector1 : Selector  IndexMode=Zero-based  InputPortWidth=16  IndexOptions=Index vector (dialog)  Indices=[6]  OutputSizes=1
  Selector6 : Selector  IndexMode=Zero-based  InputPortWidth=16  IndexOptions=Index vector (dialog)  Indices=[7]  OutputSizes=1
  Selector7 : Selector  IndexMode=Zero-based  InputPortWidth=16  IndexOptions=Index vector (dialog)  Indices=[8]  OutputSizes=1
  Selector8 : Selector  IndexMode=Zero-based  InputPortWidth=16  IndexOptions=Index vector (dialog)  Indices=[9]  OutputSizes=1
  Switch : Switch  Criteria=u2 ~= 0  InputSameDT=on
  Terminator1 : Terminator
  Terminator2 : Terminator
  Terminator3 : Terminator
  Unit Delay{,1..14} (15 alike) : UnitDelay  SampleTime=-1  HasFrameUpgradeWarning=on
  VH_usAvgVehicleSpeed : Outport  OutDataTypeStr=fixdt(0,16,0.01,0)  SampleTime=STEP_TIME  VectorParamsAs1DForOutWhenUnconnected=off
  VH_usSpeedPulseData : Outport  Port=2  OutDataTypeStr=fixdt(0,16,0.01,0)  SampleTime=STEP_TIME  VectorParamsAs1DForOutWhenUnconnected=off
  wires:
  GB_bIgn1/1 -> Terminator2/1
  IH_ucVehicleSpeedStatus/1 -> Terminator1/1
  IH_ucSpeedPulseStatus/1 -> Terminator3/1
  Mux/1 -> HeapSort/1(yLineArr)
  Unit Delay3/1 -> Mux/5, Unit Delay4/1
  Unit Delay11/1 -> Mux/13, Unit Delay12/1
  Unit Delay6/1 -> Mux/8, Unit Delay7/1
  Unit Delay2/1 -> Unit Delay3/1, Mux/4
  Unit Delay4/1 -> Mux/6, Unit Delay5/1
  Unit Delay5/1 -> Unit Delay6/1, Mux/7
  Unit Delay8/1 -> Unit Delay9/1, Mux/10
  Unit Delay12/1 -> Mux/14, Unit Delay13/1
  Unit Delay1/1 -> Unit Delay2/1, Mux/3
  Unit Delay9/1 -> Mux/11, Unit Delay10/1
  Unit Delay7/1 -> Unit Delay8/1, Mux/9
  Unit Delay10/1 -> Mux/12, Unit Delay11/1
  Unit Delay13/1 -> Mux/15, Unit Delay14/1
  Unit Delay/1 -> Unit Delay1/1, Mux/2
  Unit Delay14/1 -> Mux/16
  IH_usVehicleSpeed/1 -> Mux/1, Unit Delay/1
  Data Type Conversion1/1 -> Relational Operator/2
  Data Type Conversion3/1 -> Divide1/2
  Data Type Conversion2/1 -> Switch/1
  IH_ucSMCUT/1 -> Data Type Conversion1/1
  Switch/1 -> VH_usAvgVehicleSpeed/1
  Relational Operator/1 -> Switch/2
  Selector1/1 -> Add1/1
  Selector6/1 -> Add1/2
  Selector8/1 -> Add1/4
  Selector7/1 -> Add1/3
  Add1/1 -> Divide1/1
  Divide1/1 -> Switch/3, Relational Operator/1
  HeapSort/1(K) -> Selector1/1, Selector6/1, Selector7/1, Selector8/1
  Constant3/1 -> Data Type Conversion3/1
  Constant1/1 -> Data Type Conversion2/1
  IH_usSpeedPulse/1 -> VH_usSpeedPulseData/1

== system Speedmeter_harness/Test Unit (copied from Speedmeter)/SWC_SpeedMeter/SWC_SpeedMeter/Spd_Pointer ==
  IH_usSMV : Inport  PortDimensions=13  SampleTime=STEP_TIME
  IH_usSMD : Inport  Port=2  PortDimensions=13  SampleTime=STEP_TIME
  IH_ucADJ_SMD : Inport  Port=3  PortDimensions=13  SampleTime=STEP_TIME
  VH_usAvgVehicleSpeed : Inport  Port=4  SampleTime=STEP_TIME
  IH_ucSMCANCEL : Inport  Port=5  SampleTime=STEP_TIME
  IH_usSMDEGLIM : Inport  Port=6  SampleTime=STEP_TIME
  IH_usSMSTPLIM : Inport  Port=7  SampleTime=STEP_TIME
  IH_ucSMFILT : Inport  Port=8  OutDataTypeStr=fixdt(0,8,1,0)  SampleTime=STEP_TIME
  IH_ucSMFILT2 : Inport  Port=9  OutDataTypeStr=fixdt(0,8,1,0)  SampleTime=STEP_TIME
  IH_ucMOVE01 : Inport  Port=10  OutDataTypeStr=fixdt(0,8,1,0)  SampleTime=STEP_TIME
  IH_uc01DATA : Inport  Port=11  OutDataTypeStr=fixdt(0,8,1,0)  SampleTime=STEP_TIME
  DialOffsetProccess : Subsystem  TreatAsAtomicUnit=on
  Filter : Subsystem  TreatAsAtomicUnit=on
  InputLimitProccess : Subsystem  TreatAsAtomicUnit=on
  PointerAngleCalculation : Subsystem  TreatAsAtomicUnit=on
  Terminator : Terminator
  Terminator1 : Terminator
  OH_usSpdPtrAngle : Outport  SampleTime=STEP_TIME  VectorParamsAs1DForOutWhenUnconnected=off
  wires:
  IH_ucMOVE01/1 -> Terminator/1
  IH_uc01DATA/1 -> Terminator1/1
  InputLimitProccess/1(Dx) -> Filter/3(Dx)
  IH_ucSMFILT2/1 -> Filter/2(IH_ucSMFILT2)
  IH_ucADJ_SMD/1 -> PointerAngleCalculation/3(IH_ucADJ_SMD)
  IH_usSMD/1 -> PointerAngleCalculation/2(IH_usSMD)
  PointerAngleCalculation/1(PointerAngle) -> DialOffsetProccess/3(PointerAngle)
  VH_usAvgVehicleSpeed/1 -> PointerAngleCalculation/4(VH_usAvgVehicleSpeed)
  Filter/1(Dn2) -> OH_usSpdPtrAngle/1
  IH_ucSMFILT/1 -> Filter/1(IH_ucSMFILT)
  DialOffsetProccess/1(DA) -> InputLimitProccess/2(DA)
  IH_usSMV/1 -> PointerAngleCalculation/1(IH_usSMV)
  IH_ucSMCANCEL/1 -> DialOffsetProccess/1(IH_ucSMCANCEL)
  IH_usSMSTPLIM/1 -> InputLimitProccess/1(IH_usSMSTPLIM)
  IH_usSMDEGLIM/1 -> DialOffsetProccess/2(IH_usSMDEGLIM), Filter/4(IH_usSMDEGLIM)

== system Speedmeter_harness/Test Unit (copied from Speedmeter)/SWC_SpeedMeter/SWC_SpeedMeter/Spd_disp ==
  VH_usAvgVehicleSpeed : Inport  SampleTime=STEP_TIME
  IH_ucSMFILT : Inport  Port=2  OutDataTypeStr=fixdt(0,8,1,0)  SampleTime=STEP_TIME
  IH_ucSMFILT2 : Inport  Port=3  OutDataTypeStr=fixdt(0,8,1,0)  SampleTime=STEP_TIME
  OH_ucSetUnitSpeed : Inport  Port=4  OutDataTypeStr=fixdt(0,8,1,0)  SampleTime=STEP_TIME
  Displayfilter : Subsystem  TreatAsAtomicUnit=on
  FilteringProcess : Subsystem  TreatAsAtomicUnit=on
  UnitConversion : Subsystem  TreatAsAtomicUnit=on
  OH_usSpdDisplay : Outport  VectorParamsAs1DForOutWhenUnconnected=off
  wires:
  VH_usAvgVehicleSpeed/1 -> FilteringProcess/1(VH_usAvgVehicleSpeed)
  UnitConversion/1(Measured_V) -> [Measured_V]
  IH_ucSMFILT/1 -> FilteringProcess/2(IH_ucSMFILT)
  IH_ucSMFILT2/1 -> FilteringProcess/3(IH_ucSMFILT2)
  [Dn2] -> UnitConversion/2(Dn2)
  [Measured_V] -> Displayfilter/1(Measured_V)
  FilteringProcess/1(Dn2) -> [Dn2]
  OH_ucSetUnitSpeed/1 -> UnitConversion/1(OH_ucSetUnitSpeed)
  Displayfilter/1(OH_usSpdDisplay) -> OH_usSpdDisplay/1

== system Speedmeter_harness/Test Unit (copied from Speedmeter)/SWC_SpeedMeter/SWC_SpeedMeter/Spd_pulse ==
  VH_usSpeedPulseData : Inport  OutDataTypeStr=fixdt(0,16,0.01,0)  SampleTime=STEP_TIME
  Constant1 : Constant  Value=Const16_2  OutDataTypeStr=Inherit: Inherit via back propagation  SampleTime=STEP_TIME
  Constant10 : Constant  Value=Const16_350  OutDataTypeStr=Inherit: Inherit via back propagation  SampleTime=STEP_TIME
  Constant11 : Constant  Value=Const16_350  OutDataTypeStr=Inherit: Inherit via back propagation  SampleTime=STEP_TIME
  Constant2 : Constant  Value=Const16_0  OutDataTypeStr=Inherit: Inherit via back propagation  SampleTime=STEP_TIME
  Relational Operator1 : RelationalOperator  Operator=<  OutDataTypeStr=boolean  RndMeth=Simplest  InputSameDT=on
  Relational Operator3 : RelationalOperator  Operator=>  OutDataTypeStr=boolean  RndMeth=Simplest  InputSameDT=on
  Switch1 : Switch  Criteria=u2 ~= 0  InputSameDT=on
  Switch3 : Switch  Criteria=u2 ~= 0  InputSameDT=on
  OH_usSpd8pOut : Outport  OutDataTypeStr=fixdt(0,16,0.01,0)  SampleTime=STEP_TIME  VectorParamsAs1DForOutWhenUnconnected=off
  wires:
  Constant11/1 -> Switch3/1
  Constant10/1 -> Relational Operator3/2
  Constant2/1 -> Switch1/1
  Constant1/1 -> Relational Operator1/2
  Switch3/1 -> OH_usSpd8pOut/1
  Switch1/1 -> Switch3/3
  Relational Operator1/1 -> Switch1/2
  VH_usSpeedPulseData/1 -> Switch1/3, Relational Operator1/1, Relational Operator3/1
  Relational Operator3/1 -> Switch3/2

== system Speedmeter_harness/Test Unit (copied from Speedmeter)/SWC_SpeedMeter/SWC_SpeedMeter/Spd_Pointer/DialOffsetProccess ==
  IH_ucSMCANCEL : Inport  SampleTime=STEP_TIME
  IH_usSMDEGLIM : Inport  Port=2  SampleTime=STEP_TIME
  PointerAngle : Inport  Port=3  OutDataTypeStr=fixdt(1,32,0.0001,0)  SampleTime=STEP_TIME
  Constant : Constant  Value=ConstFL_03516  OutDataTypeStr=fixdt(0,32,0.0001,0)  SampleTime=STEP_TIME
  Constant2 : Constant  Value=Const16_0  SampleTime=STEP_TIME
  Constant3 : Constant  Value=ConstFL_03516  OutDataTypeStr=fixdt(1,32,0.0001,0)  SampleTime=STEP_TIME
  Data Type Conversion : DataTypeConversion
  Data Type Conversion5 : DataTypeConversion
  Data Type Conversion6 : DataTypeConversion
  Product : Product  OutDataTypeStr=fixdt(1,32,0.0001,0)  InputSameDT=on
  Product1 : Product  OutDataTypeStr=fixdt(1,32,0.0001,0)  InputSameDT=on
  Relational Operator1 : RelationalOperator  OutDataTypeStr=boolean  RndMeth=Simplest  InputSameDT=on
  Relational Operator2 : RelationalOperator  Operator=>  OutDataTypeStr=boolean  RndMeth=Simplest  InputSameDT=on
  Subtract : Sum  Inputs=+-  InputSameDT=on
  Switch1 : Switch  Criteria=u2 ~= 0  InputSameDT=on
  Switch2 : Switch  Criteria=u2 ~= 0  InputSameDT=on
  DA : Outport  SampleTime=STEP_TIME  VectorParamsAs1DForOutWhenUnconnected=off
  wires:
  Switch2/1 -> DA/1
  Data Type Conversion/1 -> Product/1
  IH_usSMDEGLIM/1 -> Data Type Conversion6/1
  IH_ucSMCANCEL/1 -> Data Type Conversion/1
  Relational Operator2/1 -> Switch2/2
  Switch1/1 -> Relational Operator2/1, Switch2/3
  Data Type Conversion5/1 -> Switch1/3
  Data Type Conversion6/1 -> Product1/1
  PointerAngle/1 -> Relational Operator1/1, Subtract/1
  Product/1 -> Relational Operator1/2, Subtract/2
  Relational Operator1/1 -> Switch1/2
  Constant/1 -> Product/2
  Product1/1 -> Relational Operator2/2, Switch2/1
  Constant2/1 -> Data Type Conversion5/1
  Subtract/1 -> Switch1/1
  Constant3/1 -> Product1/2
